simulink model "Test2_2"  (R2021a)
(part 3 of 3)

  Line 71 : spsDistributedParametersLineLib/Distributed Parameters Line  Phases=3  Length=0.16999  Frequency=50  Resistance=[0.646656091154803 0.0486237908083191 0.0486712220507153;0.0486237908083191 0.646561225344642 0.0486237934466192;0.0486712220507153 0.0486237934466192 0.646656091154803]  Inductance=[0.00282448912315926 0.00133270803418135 0.00132951476746136;0.00133270803418135 0.00282479813276775 0.00133799988507366;0.00132951476746136 0.00133799988507366 0.00282448912315926]  Capacitance=[7.89543174552926e-09 -1.85986777702161e-09 -1.7901190036642e-09;-1.85986777702161e-09 7.82540023894543e-09 -1.8957321828871e-09;-1.7901190036642e-09 -1.8957321828871e-09 7.91264394645417e-09]  x1=[130.230707636067 9966.01246212464 9965.41426921905;314.159265358979 314.159265358979 314.159265358979;1.01292996287477 -0.183692598773052 -1.7546536630313]  x2=[130.231666358781 9965.86534817877 9965.2673720638;314.159265358979 314.159265358979 314.159265358979;1.01293460745813 -0.183698024049707 -1.75465903275388]  x3=[0.11680712246644 24.2072409105011 24.4001350687789;314.159265358979 314.159265358979 314.159265358979;0.99559201404185 -0.16833311922206 -1.73942871924422]  x4=[0.110940912518223 26.5128987572226 26.7063295888185;314.159265358979 314.159265358979 314.159265358979;1.03092689690365 -0.197915914084497 -1.76876362475642]  x5=8.14502446416769e-07  V1=ones(3,3)  V2=ones(3,3)  I1=ones(3,3)  I2=ones(3,3)  nHarmo=1  Measurements=None  Decoupling=off  VsMag0=0  VrMag0=0  VsAngle0=0  VrAngle0=0  IsMag0=0  IrMag0=0  IsAngle0=0  IrAngle0=0
      settings: SourceProductBaseCode=PS
  Line 72 : spsDistributedParametersLineLib/Distributed Parameters Line  Phases=3  Length=0.27999  Frequency=50  Resistance=[0.646656091154803 0.0486237908083191 0.0486712220507153;0.0486237908083191 0.646561225344642 0.0486237934466192;0.0486712220507153 0.0486237934466192 0.646656091154803]  Inductance=[0.00282448912315926 0.00133270803418135 0.00132951476746136;0.00133270803418135 0.00282479813276775 0.00133799988507366;0.00132951476746136 0.00133799988507366 0.00282448912315926]  Capacitance=[7.89543174552926e-09 -1.85986777702161e-09 -1.7901190036642e-09;-1.85986777702161e-09 7.82540023894543e-09 -1.8957321828871e-09;-1.7901190036642e-09 -1.8957321828871e-09 7.91264394645417e-09]  x1=[130.081348911455 9976.99844767141 9976.35824041174;314.159265358979 314.159265358979 314.159265358979;1.01268721771526 -0.183283432469296 -1.75424455593335]  x2=[130.230707636067 9966.01246212464 9965.41426921905;314.159265358979 314.159265358979 314.159265358979;1.01276438146455 -0.183824142328408 -1.75478533180681]  x3=[0.351945699224796 33.0670710232444 32.8199427170776;314.159265358979 314.159265358979 314.159265358979;0.207747752541117 2.58745975030086 1.0223784525399]  x4=[0.254167918835229 82.4346919282585 82.619054469803;314.159265358979 314.159265358979 314.159265358979;2.64798945434631 -0.329445271930397 -1.89678242777258]  x5=1.341564444804e-06  V1=ones(3,3)  V2=ones(3,3)  I1=ones(3,3)  I2=ones(3,3)  nHarmo=1  Measurements=None  Decoupling=off  VsMag0=0  VrMag0=0  VsAngle0=0  VrAngle0=0  IsMag0=0  IrMag0=0  IsAngle0=0  IrAngle0=0
      settings: SourceProductBaseCode=PS
  Line 73 : spsDistributedParametersLineLib/Distributed Parameters Line  Phases=3  Length=0.01  Frequency=50  Resistance=[0.646656091154803 0.0486237908083191 0.0486712220507153;0.0486237908083191 0.646561225344642 0.0486237934466192;0.0486712220507153 0.0486237934466192 0.646656091154803]  Inductance=[0.00282448912315926 0.00133270803418135 0.00132951476746136;0.00133270803418135 0.00282479813276775 0.00133799988507366;0.00132951476746136 0.00133799988507366 0.00282448912315926]  Capacitance=[7.89543174552926e-09 -1.85986777702161e-09 -1.7901190036642e-09;-1.85986777702161e-09 7.82540023894543e-09 -1.8957321828871e-09;-1.7901190036642e-09 -1.8957321828871e-09 7.91264394645417e-09]  x1=[130.076014067588 9977.39085152671 9976.74914367271;314.159265358979 314.159265358979 314.159265358979;1.01309087195348 -0.182941272422882 -1.75390208607958]  x2=[130.081348911455 9976.9984476714 9976.35824041174;314.159265358979 314.159265358979 314.159265358979;1.0130936297602 -0.182960564791928 -1.75392138090882]  x3=[0.351978223037803 33.0705703263258 32.8233930888697;314.159265358979 314.159265358979 314.159265358979;0.208150829615969 2.58773785503595 1.02265661264299]  x4=[0.254237413967942 82.4786371856206 82.663380177016;314.159265358979 314.159265358979 314.159265358979;2.64887893860995 -0.328802030937441 -1.89613838575731]  x5=4.79147271261115e-08  V1=ones(3,3)  V2=ones(3,3)  I1=ones(3,3)  I2=ones(3,3)  nHarmo=1  Measurements=None  Decoupling=off  VsMag0=0  VrMag0=0  VsAngle0=0  VrAngle0=0  IsMag0=0  IrMag0=0  IsAngle0=0  IrAngle0=0
      settings: SourceProductBaseCode=PS
  Line 74 : spsDistributedParametersLineLib/Distributed Parameters Line  Phases=3  Length=0.04  Frequency=50  Resistance=[0.646656091154803 0.0486237908083191 0.0486712220507153;0.0486237908083191 0.646561225344642 0.0486237934466192;0.0486712220507153 0.0486237934466192 0.646656091154803]  Inductance=[0.00282448912315926 0.00133270803418135 0.00132951476746136;0.00133270803418135 0.00282479813276775 0.00133799988507366;0.00132951476746136 0.00133799988507366 0.00282448912315926]  Capacitance=[7.89543174552926e-09 -1.85986777702161e-09 -1.7901190036642e-09;-1.85986777702161e-09 7.82540023894543e-09 -1.8957321828871e-09;-1.7901190036642e-09 -1.8957321828871e-09 7.91264394645417e-09]  x1=[130.054674407228 9978.96048980824 9978.31277955769;314.159265358979 314.159265358979 314.159265358979;1.01303468087487 -0.182899991815375 -1.75386082971175]  x2=[130.076014067588 9977.39085152672 9976.74914367271;314.159265358979 314.159265358979 314.159265358979;1.01304571338706 -0.182977147937979 -1.75393799574563]  x3=[0.351967320325577 33.0666328859275 32.8194352751504;314.159265358979 314.159265358979 314.159265358979;0.208050372349346 2.58764038125158 1.02255895809718]  x4=[0.254236673448409 82.4773408673841 82.6620672276254;314.159265358979 314.159265358979 314.159265358979;2.6488539053286 -0.328827139194275 -1.89616350237567]  x5=1.91658908504446e-07  V1=ones(3,3)  V2=ones(3,3)  I1=ones(3,3)  I2=ones(3,3)  nHarmo=1  Measurements=None  Decoupling=off  VsMag0=0  VrMag0=0  VsAngle0=0  VrAngle0=0  IsMag0=0  IrMag0=0  IsAngle0=0  IrAngle0=0
      settings: SourceProductBaseCode=PS
  Line 75 : spsDistributedParametersLineLib/Distributed Parameters Line  Phases=3  Length=0.23  Frequency=50  Resistance=[0.646656091154803 0.0486237908083191 0.0486712220507153;0.0486237908083191 0.646561225344642 0.0486237934466192;0.0486712220507153 0.0486237934466192 0.646656091154803]  Inductance=[0.00282448912315926 0.00133270803418135 0.00132951476746136;0.00133270803418135 0.00282479813276775 0.00133799988507366;0.00132951476746136 0.00133799988507366 0.00282448912315926]  Capacitance=[7.89543174552926e-09 -1.85986777702161e-09 -1.7901190036642e-09;-1.85986777702161e-09 7.82540023894543e-09 -1.8957321828871e-09;-1.7901190036642e-09 -1.8957321828871e-09 7.91264394645417e-09]  x1=[132.412260404274 9804.45058362649 9804.44542068226;314.159265358979 314.159265358979 314.159265358979;1.01400079471883 -0.191512094576426 -1.76247536456498]  x2=[132.463644567909 9800.85070742944 9800.85908991131;314.159265358979 314.159265358979 314.159265358979;1.01403095544799 -0.191682957837417 -1.76264642626444]  x3=[0.201444563725322 5.91804966428605 5.9047215966924;314.159265358979 314.159265358979 314.159265358979;0.461275939437241 0.877082063076161 -0.728437900325085]  x4=[0.121619568555495 47.317972952253 47.5167935580992;314.159265358979 314.159265358979 314.159265358979;2.06777818856542 -0.301596093803467 -1.86970736913679]  x5=1.10203872390056e-06  V1=ones(3,3)  V2=ones(3,3)  I1=ones(3,3)  I2=ones(3,3)  nHarmo=1  Measurements=None  Decoupling=off  VsMag0=0  VrMag0=0  VsAngle0=0  VrAngle0=0  IsMag0=0  IrMag0=0  IsAngle0=0  IrAngle0=0
      settings: SourceProductBaseCode=PS
  Line 76 : spsDistributedParametersLineLib/Distributed Parameters Line  Phases=3  Length=1.62  Frequency=50  Resistance=[0.80718830189013 0.0486237908083191 0.0486712220507153;0.0486237908083191 0.807093436079969 0.0486237934466192;0.0486712220507153 0.0486237934466192 0.80718830189013]  Inductance=[0.00279786707424938 0.00133270803418135 0.00132951476746136;0.00133270803418135 0.00279817608385787 0.00133799988507366;0.00132951476746136 0.00133799988507366 0.00279786707424938]  Capacitance=[7.73340098830622e-09 -1.79942827973291e-09 -1.73218055098733e-09;-1.79942827973291e-09 7.66505189233746e-09 -1.83375898618858e-09;-1.73218055098733e-09 -1.83375898618858e-09 7.749673531177e-09]  x1=[55.945966993339 9804.5358454258 9804.6105183802;314.159265358979 314.159265358979 314.159265358979;1.07738009221999 -0.197446923817235 -1.76837194176404]  x2=[55.9463733224315 9804.53267731463 9804.60740490844;314.159265358979 314.159265358979 314.159265358979;1.07738098322596 -0.197450312552494 -1.76837534864892]  x3=[0.048782988865129 24.8163020226173 25.0053176417309;314.159265358979 314.159265358979 314.159265358979;1.07397701542993 -0.199145104328598 -1.77007334483569]  x4=[0.0486344229699074 24.8439993842728 25.0330218787076;314.159265358979 314.159265358979 314.159265358979;1.07836957224309 -0.197652494246344 -1.76857592031423]  x5=7.70442045759223e-06  V1=ones(3,3)  V2=ones(3,3)  I1=ones(3,3)  I2=ones(3,3)  nHarmo=1  Measurements=None  Decoupling=off  VsMag0=0  VrMag0=0  VsAngle0=0  VrAngle0=0  IsMag0=0  IrMag0=0  IsAngle0=0  IrAngle0=0
      settings: SourceProductBaseCode=PS
  Line 77 : spsDistributedParametersLineLib/Distributed Parameters Line  Phases=3  Length=0.54002  Frequency=50  Resistance=[0.646656091154803 0.0486237908083191 0.0486712220507153;0.0486237908083191 0.646561225344642 0.0486237934466192;0.0486712220507153 0.0486237934466192 0.646656091154803]  Inductance=[0.00282448912315926 0.00133270803418135 0.00132951476746136;0.00133270803418135 0.00282479813276775 0.00133799988507366;0.00132951476746136 0.00133799988507366 0.00282448912315926]  Capacitance=[7.89543174552926e-09 -1.85986777702161e-09 -1.7901190036642e-09;-1.85986777702161e-09 7.82540023894543e-09 -1.8957321828871e-09;-1.7901190036642e-09 -1.8957321828871e-09 7.91264394645417e-09]  x1=[132.291266816328 9812.89477090012 9812.85777166442;314.159265358979 314.159265358979 314.159265358979;1.01346404772917 -0.191480026465655 -1.76244316834521]  x2=[132.412260404274 9804.45058362648 9804.44542068226;314.159265358979 314.159265358979 314.159265358979;1.01353412609343 -0.191882832149439 -1.76284645505391]  x3=[0.201567889892652 5.87666255876112 5.86393316817952;314.159265358979 314.159265358979 314.159265358979;0.458951197067185 0.872065549478006 -0.733742805316799]  x4=[0.121849735716523 47.3209732619761 47.5197600194276;314.159265358979 314.159265358979 314.159265358979;2.06926877558048 -0.300800439731374 -1.86890738882715]  x5=2.58749109426427e-06  V1=ones(3,3)  V2=ones(3,3)  I1=ones(3,3)  I2=ones(3,3)  nHarmo=1  Measurements=None  Decoupling=off  VsMag0=0  VrMag0=0  VsAngle0=0  VrAngle0=0  IsMag0=0  IrMag0=0  IsAngle0=0  IrAngle0=0
      settings: SourceProductBaseCode=PS
  Line 78 : spsDistributedParametersLineLib/Distributed Parameters Line  Phases=3  Length=0.13998  Frequency=50  Resistance=[0.646656091154803 0.0486237908083191 0.0486712220507153;0.0486237908083191 0.646561225344642 0.0486237934466192;0.0486712220507153 0.0486237934466192 0.646656091154803]  Inductance=[0.00282448912315926 0.00133270803418135 0.00132951476746136;0.00133270803418135 0.00282479813276775 0.00133799988507366;0.00132951476746136 0.00133799988507366 0.00282448912315926]  Capacitance=[7.89543174552926e-09 -1.85986777702161e-09 -1.7901190036642e-09;-1.85986777702161e-09 7.82540023894543e-09 -1.8957321828871e-09;-1.7901190036642e-09 -1.8957321828871e-09 7.91264394645417e-09]  x1=[132.291266816328 9812.89477090012 9812.85777166442;314.159265358979 314.159265358979 314.159265358979;1.01406622215955 -0.191001638430341 -1.76196432491836]  x2=[132.292845424718 9812.66004338261 9812.62343176244;314.159265358979 314.159265358979 314.159265358979;1.01407237967124 -0.191008438249104 -1.76197103940269]  x3=[0.12096739474067 22.8643419842892 23.0551762295825;314.159265358979 314.159265358979 314.159265358979;0.978461634859785 -0.153044666068339 -1.7243421085877]  x4=[0.110511651176818 27.1030634556416 27.2952571420408;314.159265358979 314.159265358979 314.159265358979;1.05282682069514 -0.223180765740182 -1.79390083466488]  x5=6.70710350311308e-07  V1=ones(3,3)  V2=ones(3,3)  I1=ones(3,3)  I2=ones(3,3)  nHarmo=1  Measurements=None  Decoupling=off  VsMag0=0  VrMag0=0  VsAngle0=0  VrAngle0=0  IsMag0=0  IrMag0=0  IsAngle0=0  IrAngle0=0
      settings: SourceProductBaseCode=PS
  Line 79 : spsDistributedParametersLineLib/Distributed Parameters Line  Phases=3  Length=0.14997  Frequency=50  Resistance=[0.476003738225748 0.351747138225748 0.351747138225748;0.351747138225748 0.476003738225748 0.351747138225748;0.351747138225748 0.351747138225748 0.476003738225748]  Inductance=[0.000705954362986426 0.000459934243504405 0.000459934243504405;0.000459934243504405 0.000705954362986426 0.000459934243504405;0.000459934243504405 0.000459934243504405 0.000705954362986426]  Capacitance=[5.7561313269996e-07 -1.37543883484145e-07 -1.37543912800485e-07;-1.37543883484145e-07 5.75613027339387e-07 -1.37543875208088e-07;-1.37543912800485e-07 -1.37543875208088e-07 5.75613005057695e-07]  x1=[4.71515960684011 9813.69450340501 9814.51176058105;314.159265358979 314.159265358979 314.159265358979;1.25450518806029 -0.109813676620328 -1.68063059343959]  x2=[4.71516216671498 9813.64296638232 9814.4602192662;314.159265358979 314.159265358979 314.159265358979;1.2545039381504 -0.109814213858509 -1.68063113067772]  x3=[0.0639907956313669 525.855364885648 525.899115869334;314.159265358979 314.159265358979 314.159265358979;1.25346387218607 -0.108157208623661 -1.67897412521659]  x4=[0.0639907219423131 530.093106739202 530.137210630382;314.159265358979 314.159265358979 314.159265358979;1.25450319439072 -0.112079167068294 -1.68289608406262]  x5=3.31498451375949e-06  V1=ones(3,3)  V2=ones(3,3)  I1=ones(3,3)  I2=ones(3,3)  nHarmo=1  Measurements=None  Decoupling=off  VsMag0=0  VrMag0=0  VsAngle0=0  VrAngle0=0  IsMag0=0  IrMag0=0  IsAngle0=0  IrAngle0=0
      settings: SourceProductBaseCode=PS
  Line 8 : spsDistributedParametersLineLib/Distributed Parameters Line  Phases=3  Length=0.54002  Frequency=50  Resistance=[0.646656091154803 0.0486237908083191 0.0486712220507153;0.0486237908083191 0.646561225344642 0.0486237934466192;0.0486712220507153 0.0486237934466192 0.646656091154803]  Inductance=[0.00282448912315926 0.00133270803418135 0.00132951476746136;0.00133270803418135 0.00282479813276775 0.00133799988507366;0.00132951476746136 0.00133799988507366 0.00282448912315926]  Capacitance=[7.89543174552926e-09 -1.85986777702161e-09 -1.7901190036642e-09;-1.85986777702161e-09 7.82540023894543e-09 -1.8957321828871e-09;-1.7901190036642e-09 -1.8957321828871e-09 7.91264394645417e-09]  x1=[131.737607363178 9850.69941802642 9850.17864308144;314.159265358979 314.159265358979 314.159265358979;1.06906824241826 2.25892076126052 -2.45322280325767]  x2=[131.749735782929 9848.86865393328 9848.36073374528;314.159265358979 314.159265358979 314.159265358979;1.06911835002861 2.25882438625055 -2.45331782899078]  x3=[0.126165540353935 20.1433647221107 20.3624969468267;314.159265358979 314.159265358979 314.159265358979;1.00194096644596 2.30506910238496 -2.40791035448599]  x4=[0.104769515257823 29.9954148200453 30.1573900029457;314.159265358979 314.159265358979 314.159265358979;1.14909044449937 2.22731573734265 -2.48443339458061]  x5=2.58749109426427e-06  V1=ones(3,3)  V2=ones(3,3)  I1=ones(3,3)  I2=ones(3,3)  nHarmo=1  Measurements=None  Decoupling=off  VsMag0=0  VrMag0=0  VsAngle0=0  VrAngle0=0  IsMag0=0  IrMag0=0  IsAngle0=0  IrAngle0=0
      settings: SourceProductBaseCode=PS
  Line 80 : spsDistributedParametersLineLib/Distributed Parameters Line  Phases=3  Length=0.50001  Frequency=50  Resistance=[0.646656091154803 0.0486237908083191 0.0486712220507153;0.0486237908083191 0.646561225344642 0.0486237934466192;0.0486712220507153 0.0486237934466192 0.646656091154803]  Inductance=[0.00282448912315926 0.00133270803418135 0.00132951476746136;0.00133270803418135 0.00282479813276775 0.00133799988507366;0.00132951476746136 0.00133799988507366 0.00282448912315926]  Capacitance=[7.89543174552926e-09 -1.85986777702161e-09 -1.7901190036642e-09;-1.85986777702161e-09 7.82540023894543e-09 -1.8957321828871e-09;-1.7901190036642e-09 -1.8957321828871e-09 7.91264394645417e-09]  x1=[132.173511194652 9821.5491506484 9821.48128373896;314.159265358979 314.159265358979 314.159265358979;1.0134375447102 -0.191035064587028 -1.76199801385489]  x2=[132.291266816328 9812.89477090012 9812.85777166442;314.159265358979 314.159265358979 314.159265358979;1.01352427420392 -0.191432180487021 -1.76239527682059]  x3=[0.208251616174679 6.04681336924297 5.95781439739661;314.159265358979 314.159265358979 314.159265358979;0.454006047704687 1.25385757439675 -0.347831363027163]  x4=[0.123233192274608 49.5472322137343 49.745025795091;314.159265358979 314.159265358979 314.159265358979;2.12459359899353 -0.312913395507311 -1.88108383764282]  x5=2.3957842710327e-06  V1=ones(3,3)  V2=ones(3,3)  I1=ones(3,3)  I2=ones(3,3)  nHarmo=1  Measurements=None  Decoupling=off  VsMag0=0  VrMag0=0  VsAngle0=0  VrAngle0=0  IsMag0=0  IrMag0=0  IsAngle0=0  IrAngle0=0
      settings: SourceProductBaseCode=PS
  Line 81 : spsDistributedParametersLineLib/Distributed Parameters Line  Phases=3  Length=0.17  Frequency=50  Resistance=[0.646656091154803 0.0486237908083191 0.0486712220507153;0.0486237908083191 0.646561225344642 0.0486237934466192;0.0486712220507153 0.0486237934466192 0.646656091154803]  Inductance=[0.00282448912315926 0.00133270803418135 0.00132951476746136;0.00133270803418135 0.00282479813276775 0.00133799988507366;0.00132951476746136 0.00133799988507366 0.00282448912315926]  Capacitance=[7.89543174552926e-09 -1.85986777702161e-09 -1.7901190036642e-09;-1.85986777702161e-09 7.82540023894543e-09 -1.8957321828871e-09;-1.7901190036642e-09 -1.8957321828871e-09 7.91264394645417e-09]  x1=[132.173511194652 9821.5491506484 9821.48128373896;314.159265358979 314.159265358979 314.159265358979;1.01393430399369 -0.190640421962455 -1.76160299555848]  x2=[132.174611034258 9821.39203565152 9821.32452928868;314.159265358979 314.159265358979 314.159265358979;1.01393658179971 -0.190641437142496 -1.76160396248969]  x3=[0.117821532066125 23.996687820586 24.1879409451263;314.159265358979 314.159265358979 314.159265358979;0.990089624694144 -0.161975456637961 -1.73317290655121]  x4=[0.113355728035019 26.0018361630863 26.1938777560759;314.159265358979 314.159265358979 314.159265358979;1.03845993908498 -0.217290771556384 -1.78805201032636]  x5=8.14550361143895e-07  V1=ones(3,3)  V2=ones(3,3)  I1=ones(3,3)  I2=ones(3,3)  nHarmo=1  Measurements=None  Decoupling=off  VsMag0=0  VrMag0=0  VsAngle0=0  VrAngle0=0  IsMag0=0  IrMag0=0  IsAngle0=0  IrAngle0=0
      settings: SourceProductBaseCode=PS
  Line 82 : spsDistributedParametersLineLib/Distributed Parameters Line  Phases=3  Length=0.27998  Frequency=50  Resistance=[0.646656091154803 0.0486237908083191 0.0486712220507153;0.0486237908083191 0.646561225344642 0.0486237934466192;0.0486712220507153 0.0486237934466192 0.646656091154803]  Inductance=[0.00282448912315926 0.00133270803418135 0.00132951476746136;0.00133270803418135 0.00282479813276775 0.00133799988507366;0.00132951476746136 0.00133799988507366 0.00282448912315926]  Capacitance=[7.89543174552926e-09 -1.85986777702161e-09 -1.7901190036642e-09;-1.85986777702161e-09 7.82540023894543e-09 -1.8957321828871e-09;-1.7901190036642e-09 -1.8957321828871e-09 7.91264394645417e-09]  x1=[132.105723330459 9826.65273155558 9826.56698331564;314.159265358979 314.159265358979 314.159265358979;1.01371649706855 -0.190547975485568 -1.76151066831513]  x2=[132.173511194652 9821.5491506484 9821.48128373896;314.159265358979 314.159265358979 314.159265358979;1.01376875268919 -0.190771941600801 -1.76173464039421]  x3=[0.211636496235117 6.68880111407065 6.57085313286914;314.159265358979 314.159265358979 314.159265358979;0.448331216526076 1.41419172603944 -0.182002646191028]  x4=[0.124839280490729 50.6584149883052 50.8552864090743;314.159265358979 314.159265358979 314.159265358979;2.15192808628306 -0.323173368600227 -1.89135406139734]  x5=1.34151653007687e-06  V1=ones(3,3)  V2=ones(3,3)  I1=ones(3,3)  I2=ones(3,3)  nHarmo=1  Measurements=None  Decoupling=off  VsMag0=0  VrMag0=0  VsAngle0=0  VrAngle0=0  IsMag0=0  IrMag0=0  IsAngle0=0  IrAngle0=0
      settings: SourceProductBaseCode=PS
  Line 83 : spsDistributedParametersLineLib/Distributed Parameters Line  Phases=3  Length=0.03  Frequency=50  Resistance=[0.476003738225748 0.351747138225748 0.351747138225748;0.351747138225748 0.476003738225748 0.351747138225748;0.351747138225748 0.351747138225748 0.476003738225748]  Inductance=[0.000705954362986426 0.000459934243504405 0.000459934243504405;0.000459934243504405 0.000705954362986426 0.000459934243504405;0.000459934243504405 0.000459934243504405 0.000705954362986426]  Capacitance=[5.7561313269996e-07 -1.37543883484145e-07 -1.37543912800485e-07;-1.37543883484145e-07 5.75613027339387e-07 -1.37543875208088e-07;-1.37543912800485e-07 -1.37543875208088e-07 5.75613005057695e-07]  x1=[5.70282059813818 9777.61614892348 9777.73874302418;314.159265358979 314.159265358979 314.159265358979;1.28263867287871 2.17477579081481 -2.53751546513187]  x2=[5.70282402151544 9777.6163039351 9777.73889895204;314.159265358979 314.159265358979 314.159265358979;1.28263665860042 2.17477576530025 -2.53751549074301]  x3=[0.0774700274359414 526.350277214598 526.356899317948;314.159265358979 314.159265358979 314.159265358979;1.27855129628944 2.17458627167104 -2.53770554021627]  x4=[0.0775438111432303 526.350340456895 526.35683612321;314.159265358979 314.159265358979 314.159265358979;1.28651189534568 2.17484043953016 -2.53745026053335]  x5=6.63129528657629e-07  V1=ones(3,3)  V2=ones(3,3)  I1=ones(3,3)  I2=ones(3,3)  nHarmo=1  Measurements=None  Decoupling=off  VsMag0=0  VrMag0=0  VsAngle0=0  VrAngle0=0  IsMag0=0  IrMag0=0  IsAngle0=0  IrAngle0=0
      settings: SourceProductBaseCode=PS
  Line 84 : spsDistributedParametersLineLib/Distributed Parameters Line  Phases=3  Length=0.02  Frequency=50  Resistance=[0.646656091154803 0.0486237908083191 0.0486712220507153;0.0486237908083191 0.646561225344642 0.0486237934466192;0.0486712220507153 0.0486237934466192 0.646656091154803]  Inductance=[0.00282448912315926 0.00133270803418135 0.00132951476746136;0.00133270803418135 0.00282479813276775 0.00133799988507366;0.00132951476746136 0.00133799988507366 0.00282448912315926]  Capacitance=[7.89543174552926e-09 -1.85986777702161e-09 -1.7901190036642e-09;-1.85986777702161e-09 7.82540023894543e-09 -1.8957321828871e-09;-1.7901190036642e-09 -1.8957321828871e-09 7.91264394645417e-09]  x1=[132.789126266165 9781.02683598408 9780.42031592206;314.159265358979 314.159265358979 314.159265358979;1.0694910373007 2.25677854886239 -2.45535788755353]  x2=[132.789137662631 9781.02358008288 9780.417064447;314.159265358979 314.159265358979 314.159265358979;1.06949120331148 2.25677843562566 -2.45535799936825]  x3=[0.116761225704046 24.6778683791443 24.8674778921864;314.159265358979 314.159265358979 314.159265358979;1.06907973129993 2.25980703976288 -2.45234982662511]  x4=[0.115440893096846 25.1044925257125 25.2941175783022;314.159265358979 314.159265358979 314.159265358979;1.06987693711702 2.25377769785739 -2.45833905984952]  x5=9.5829454252223e-08  V1=ones(3,3)  V2=ones(3,3)  I1=ones(3,3)  I2=ones(3,3)  nHarmo=1  Measurements=None  Decoupling=off  VsMag0=0  VrMag0=0  VsAngle0=0  VrAngle0=0  IsMag0=0  IrMag0=0  IsAngle0=0  IrAngle0=0
      settings: SourceProductBaseCode=PS
  Line 85 : spsDistributedParametersLineLib/Distributed Parameters Line  Phases=3  Length=0.5  Frequency=50  Resistance=[0.646656091154803 0.0486237908083191 0.0486712220507153;0.0486237908083191 0.646561225344642 0.0486237934466192;0.0486712220507153 0.0486237934466192 0.646656091154803]  Inductance=[0.00282448912315926 0.00133270803418135 0.00132951476746136;0.00133270803418135 0.00282479813276775 0.00133799988507366;0.00132951476746136 0.00133799988507366 0.00282448912315926]  Capacitance=[7.89543174552926e-09 -1.85986777702161e-09 -1.7901190036642e-09;-1.85986777702161e-09 7.82540023894543e-09 -1.8957321828871e-09;-1.7901190036642e-09 -1.8957321828871e-09 7.91264394645417e-09]  x1=[132.772277667242 9782.18789453562 9781.57741920365;314.159265358979 314.159265358979 314.159265358979;1.06865004930001 2.25627362822203 -2.45586345652191]  x2=[132.789126266165 9781.02683598408 9780.42031592206;314.159265358979 314.159265358979 314.159265358979;1.06876850023796 2.25620454062084 -2.45593244221029]  x3=[0.138932344380155 21.3879588893918 21.5760908704784;314.159265358979 314.159265358979 314.159265358979;0.997328465291815 2.27881622397395 -2.43417244694111]  x4=[0.0940686620565523 28.3796934758062 28.569767773675;314.159265358979 314.159265358979 314.159265358979;1.17330576576078 2.23870042108029 -2.47282996263106]  x5=2.39573635630557e-06  V1=ones(3,3)  V2=ones(3,3)  I1=ones(3,3)  I2=ones(3,3)  nHarmo=1  Measurements=None  Decoupling=off  VsMag0=0  VrMag0=0  VsAngle0=0  VrAngle0=0  IsMag0=0  IrMag0=0  IsAngle0=0  IrAngle0=0
      settings: SourceProductBaseCode=PS
  Line 86 : spsDistributedParametersLineLib/Distributed Parameters Line  Phases=3  Length=0.23  Frequency=50  Resistance=[0.646656091154803 0.0486237908083191 0.0486712220507153;0.0486237908083191 0.646561225344642 0.0486237934466192;0.0486712220507153 0.0486237934466192 0.646656091154803]  Inductance=[0.00282448912315926 0.00133270803418135 0.00132951476746136;0.00133270803418135 0.00282479813276775 0.00133799988507366;0.00132951476746136 0.00133799988507366 0.00282448912315926]  Capacitance=[7.89543174552926e-09 -1.85986777702161e-09 -1.7901190036642e-09;-1.85986777702161e-09 7.82540023894543e-09 -1.8957321828871e-09;-1.7901190036642e-09 -1.8957321828871e-09 7.91264394645417e-09]  x1=[132.763119314431 9783.00719565047 9782.39424411809;314.159265358979 314.159265358979 314.159265358979;1.06899046178697 2.25663045801336 -2.4555064707107]  x2=[132.772277667242 9782.18789453562 9781.57741920365;314.159265358979 314.159265358979 314.159265358979;1.06905647639781 2.2565965078579 -2.45554026952749]  x3=[0.143597106193202 20.0832952923519 20.2705925459986;314.159265358979 314.159265358979 314.159265358979;0.98901855645717 2.32630530774299 -2.38715277073359]  x4=[0.0897348029105246 29.7768464771282 29.9663998686376;314.159265358979 314.159265358979 314.159265358979;1.19681358000998 2.20939971113767 -2.50198336508607]  x5=1.10203872390056e-06  V1=ones(3,3)  V2=ones(3,3)  I1=ones(3,3)  I2=ones(3,3)  nHarmo=1  Measurements=None  Decoupling=off  VsMag0=0  VrMag0=0  VsAngle0=0  VrAngle0=0  IsMag0=0  IrMag0=0  IsAngle0=0  IrAngle0=0
      settings: SourceProductBaseCode=PS
  Line 87 : spsDistributedParametersLineLib/Distributed Parameters Line  Phases=3  Length=1.62  Frequency=50  Resistance=[0.80718830189013 0.0486237908083191 0.0486712220507153;0.0486237908083191 0.807093436079969 0.0486237934466192;0.0486712220507153 0.0486237934466192 0.80718830189013]  Inductance=[0.00279786707424938 0.00133270803418135 0.00132951476746136;0.00133270803418135 0.00279817608385787 0.00133799988507366;0.00132951476746136 0.00133799988507366 0.00279786707424938]  Capacitance=[7.73340098830622e-09 -1.79942827973291e-09 -1.73218055098733e-09;-1.79942827973291e-09 7.66505189233746e-09 -1.83375898618858e-09;-1.73218055098733e-09 -1.83375898618858e-09 7.749673531177e-09]  x1=[56.3393685664166 9783.09162793975 9782.56182202606;314.159265358979 314.159265358979 314.159265358979;1.02643034834768 2.25931904448646 -2.45285760389577]  x2=[56.3398015731102 9783.08191094594 9782.55218276093;314.159265358979 314.159265358979 314.159265358979;1.02643301251892 2.25931608136779 -2.45286058287975]  x3=[0.0491576657452382 24.7596318145718 24.9466956947032;314.159265358979 314.159265358979 314.159265358979;1.02319452565439 2.25781599346474 -2.45436505584523]  x4=[0.0489447535654206 24.7920310467614 24.9790941839298;314.159265358979 314.159265358979 314.159265358979;1.02725646422453 2.25891888154773 -2.45325499695565]  x5=7.70442045759223e-06  V1=ones(3,3)  V2=ones(3,3)  I1=ones(3,3)  I2=ones(3,3)  nHarmo=1  Measurements=None  Decoupling=off  VsMag0=0  VrMag0=0  VsAngle0=0  VrAngle0=0  IsMag0=0  IrMag0=0  IsAngle0=0  IrAngle0=0
      settings: SourceProductBaseCode=PS
  Line 88 : spsDistributedParametersLineLib/Distributed Parameters Line  Phases=3  Length=0.54002  Frequency=50  Resistance=[0.646656091154803 0.0486237908083191 0.0486712220507153;0.0486237908083191 0.646561225344642 0.0486237934466192;0.0486712220507153 0.0486237934466192 0.646656091154803]  Inductance=[0.00282448912315926 0.00133270803418135 0.00132951476746136;0.00133270803418135 0.00282479813276775 0.00133799988507366;0.00132951476746136 0.00133799988507366 0.00282448912315926]  Capacitance=[7.89543174552926e-09 -1.85986777702161e-09 -1.7901190036642e-09;-1.85986777702161e-09 7.82540023894543e-09 -1.8957321828871e-09;-1.7901190036642e-09 -1.8957321828871e-09 7.91264394645417e-09]  x1=[132.741273272324 9784.92376829306 9784.30496184118;314.159265358979 314.159265358979 314.159265358979;1.06836945341264 2.25634143966523 -2.45579618398973]  x2=[132.763119314431 9783.00719565047 9782.39424411809;314.159265358979 314.159265358979 314.159265358979;1.06852379316157 2.25625972044035 -2.45587756119963]  x3=[0.143641248405531 20.0607836635622 20.248008773117;314.159265358979 314.159265358979 314.159265358979;0.98583218030511 2.32343330437969 -2.39002868167626]  x4=[0.0897014943316794 29.7831134823281 29.9725499420936;314.159265358979 314.159265358979 314.159265358979;1.19991552005365 2.21056085927069 -2.50081763905518]  x5=2.58749109426427e-06  V1=ones(3,3)  V2=ones(3,3)  I1=ones(3,3)  I2=ones(3,3)  nHarmo=1  Measurements=None  Decoupling=off  VsMag0=0  VrMag0=0  VsAngle0=0  VrAngle0=0  IsMag0=0  IrMag0=0  IsAngle0=0  IrAngle0=0
      settings: SourceProductBaseCode=PS
  Line 89 : spsDistributedParametersLineLib/Distributed Parameters Line  Phases=3  Length=0.13998  Frequency=50  Resistance=[0.646656091154803 0.0486237908083191 0.0486712220507153;0.0486237908083191 0.646561225344642 0.0486237934466192;0.0486712220507153 0.0486237934466192 0.646656091154803]  Inductance=[0.00282448912315926 0.00133270803418135 0.00132951476746136;0.00133270803418135 0.00282479813276775 0.00133799988507366;0.00132951476746136 0.00133799988507366 0.00282448912315926]  Capacitance=[7.89543174552926e-09 -1.85986777702161e-09 -1.7901190036642e-09;-1.85986777702161e-09 7.82540023894543e-09 -1.8957321828871e-09;-1.7901190036642e-09 -1.8957321828871e-09 7.91264394645417e-09]  x1=[132.741273272324 9784.92376829306 9784.30496184118;314.159265358979 314.159265358979 314.159265358979;1.06897162784302 2.25681982770054 -2.45531734056288]  x2=[132.742144181348 9784.70157324549 9784.08312046605;314.159265358979 314.159265358979 314.159265358979;1.06898234819054 2.25681364423754 -2.45532343075775]  x3=[0.122348512607476 22.9207989995043 23.1102774805994;314.159265358979 314.159265358979 314.159265358979;1.06151645242125 2.29351332151557 -2.41889675270657]  x4=[0.109764101877681 26.9025028907462 27.0920681426183;314.159265358979 314.159265358979 314.159265358979;1.07707009525723 2.22539834880836 -2.48654410911055]  x5=6.70710350311308e-07  V1=ones(3,3)  V2=ones(3,3)  I1=ones(3,3)  I2=ones(3,3)  nHarmo=1  Measurements=None  Decoupling=off  VsMag0=0  VrMag0=0  VsAngle0=0  VrAngle0=0  IsMag0=0  IrMag0=0  IsAngle0=0  IrAngle0=0
      settings: SourceProductBaseCode=PS
  Line 9 : spsDistributedParametersLineLib/Distributed Parameters Line  Phases=3  Length=0.13998  Frequency=50  Resistance=[0.646656091154803 0.0486237908083191 0.0486712220507153;0.0486237908083191 0.646561225344642 0.0486237934466192;0.0486712220507153 0.0486237934466192 0.646656091154803]  Inductance=[0.00282448912315926 0.00133270803418135 0.00132951476746136;0.00133270803418135 0.00282479813276775 0.00133799988507366;0.00132951476746136 0.00133799988507366 0.00282448912315926]  Capacitance=[7.89543174552926e-09 -1.85986777702161e-09 -1.7901190036642e-09;-1.85986777702161e-09 7.82540023894543e-09 -1.8957321828871e-09;-1.7901190036642e-09 -1.8957321828871e-09 7.91264394645417e-09]  x1=[131.737607363178 9850.69941802642 9850.17864308144;314.159265358979 314.159265358979 314.159265358979;1.06967041684863 2.25939914929583 -2.45274395983082]  x2=[131.738146099414 9850.54058868395 9850.0200090178;314.159265358979 314.159265358979 314.159265358979;1.06967879000639 2.25939310066086 -2.4527499382122]  x3=[0.119847205487519 23.5509521578462 23.7419853359846;314.159265358979 314.159265358979 314.159265358979;1.06772903623956 2.27977439156491 -2.43251296261474]  x4=[0.110503582508618 26.5878301855748 26.779037154267;314.159265358979 314.159265358979 314.159265358979;1.07156505501998 2.24118790525267 -2.4708439643076]  x5=6.70710350311308e-07  V1=ones(3,3)  V2=ones(3,3)  I1=ones(3,3)  I2=ones(3,3)  nHarmo=1  Measurements=None  Decoupling=off  VsMag0=0  VrMag0=0  VsAngle0=0  VrAngle0=0  IsMag0=0  IrMag0=0  IsAngle0=0  IrAngle0=0
      settings: SourceProductBaseCode=PS
  Line 90 : spsDistributedParametersLineLib/Distributed Parameters Line  Phases=3  Length=0.14997  Frequency=50  Resistance=[0.476003738225748 0.351747138225748 0.351747138225748;0.351747138225748 0.476003738225748 0.351747138225748;0.351747138225748 0.351747138225748 0.476003738225748]  Inductance=[0.000705954362986426 0.000459934243504405 0.000459934243504405;0.000459934243504405 0.000705954362986426 0.000459934243504405;0.000459934243504405 0.000459934243504405 0.000705954362986426]  Capacitance=[5.7561313269996e-07 -1.37543883484145e-07 -1.37543912800485e-07;-1.37543883484145e-07 5.75613027339387e-07 -1.37543875208088e-07;-1.37543912800485e-07 -1.37543875208088e-07 5.75613005057695e-07]  x1=[3.62838796694639 9851.63719589281 9851.85858599348;314.159265358979 314.159265358979 314.159265358979;1.30289632755562 2.17728914964739 -2.53500824297292]  x2=[3.62838993117416 9851.60136193109 9851.82275122619;314.159265358979 314.159265358979 314.159265358979;1.30289507320158 2.17728859167297 -2.53500880094729]  x3=[0.0492418432482476 528.498059284221 528.509894969357;314.159265358979 314.159265358979 314.159265358979;1.30185368891968 2.17820493731586 -2.53409245513826]  x4=[0.0492419064510967 531.532638855963 531.544542736239;314.159265358979 314.159265358979 314.159265358979;1.30289564998328 2.17575559094808 -2.53654180178885]  x5=3.31498451375949e-06  V1=ones(3,3)  V2=ones(3,3)  I1=ones(3,3)  I2=ones(3,3)  nHarmo=1  Measurements=None  Decoupling=off  VsMag0=0  VrMag0=0  VsAngle0=0  VrAngle0=0  IsMag0=0  IrMag0=0  IsAngle0=0  IrAngle0=0
      settings: SourceProductBaseCode=PS
  Line 91 : spsDistributedParametersLineLib/Distributed Parameters Line  Phases=3  Length=0.50001  Frequency=50  Resistance=[0.646656091154803 0.0486237908083191 0.0486712220507153;0.0486237908083191 0.646561225344642 0.0486237934466192;0.0486712220507153 0.0486237934466192 0.646656091154803]  Inductance=[0.00282448912315926 0.00133270803418135 0.00132951476746136;0.00133270803418135 0.00282479813276775 0.00133799988507366;0.00132951476746136 0.00133799988507366 0.00282448912315926]  Capacitance=[7.89543174552926e-09 -1.85986777702161e-09 -1.7901190036642e-09;-1.85986777702161e-09 7.82540023894543e-09 -1.8957321828871e-09;-1.7901190036642e-09 -1.8957321828871e-09 7.91264394645417e-09]  x1=[131.72436565465 9852.95782936429 9852.42444400894;314.159265358979 314.159265358979 314.159265358979;1.0690524409797 2.25907994193154 -2.45306507192224]  x2=[131.737607363178 9850.69941802642 9850.17864308144;314.159265358979 314.159265358979 314.159265358979;1.06912846889301 2.25896860723915 -2.45317491173305]  x3=[0.130839345427691 18.6625362785029 18.881067013325;314.159265358979 314.159265358979 314.159265358979;1.00188876918853 2.33388258016365 -2.37947862946837]  x4=[0.100132534653049 31.5363417717655 31.6982649736186;314.159265358979 314.159265358979 314.159265358979;1.15607831111184 2.21427597413681 -2.49743613497584]  x5=2.3957842710327e-06  V1=ones(3,3)  V2=ones(3,3)  I1=ones(3,3)  I2=ones(3,3)  nHarmo=1  Measurements=None  Decoupling=off  VsMag0=0  VrMag0=0  VsAngle0=0  VrAngle0=0  IsMag0=0  IrMag0=0  IsAngle0=0  IrAngle0=0
      settings: SourceProductBaseCode=PS
  Line 92 : spsDistributedParametersLineLib/Distributed Parameters Line  Phases=3  Length=0.17  Frequency=50  Resistance=[0.646656091154803 0.0486237908083191 0.0486712220507153;0.0486237908083191 0.646561225344642 0.0486237934466192;0.0486712220507153 0.0486237934466192 0.646656091154803]  Inductance=[0.00282448912315926 0.00133270803418135 0.00132951476746136;0.00133270803418135 0.00282479813276775 0.00133799988507366;0.00132951476746136 0.00133799988507366 0.00282448912315926]  Capacitance=[7.89543174552926e-09 -1.85986777702161e-09 -1.7901190036642e-09;-1.85986777702161e-09 7.82540023894543e-09 -1.8957321828871e-09;-1.7901190036642e-09 -1.8957321828871e-09 7.91264394645417e-09]  x1=[131.72436565465 9852.95782936429 9852.42444400894;314.159265358979 314.159265358979 314.159265358979;1.06954920026319 2.25947458455612 -2.45267005362583]  x2=[131.72470187884 9852.82734590794 9852.29405478689;314.159265358979 314.159265358979 314.159265358979;1.06955685319491 2.25946763519511 -2.4526769405039]  x3=[0.118483746040794 23.9499619906877 24.1410016374452;314.159265358979 314.159265358979 314.159265358979;1.07182009354702 2.26802289386471 -2.44417671274052]  x4=[0.111840622195946 26.1910875959685 26.382330507613;314.159265358979 314.159265358979 314.159265358979;1.06688779436018 2.25145649393546 -2.46064327253397]  x5=8.14550361143895e-07  V1=ones(3,3)  V2=ones(3,3)  I1=ones(3,3)  I2=ones(3,3)  nHarmo=1  Measurements=None  Decoupling=off  VsMag0=0  VrMag0=0  VsAngle0=0  VrAngle0=0  IsMag0=0  IrMag0=0  IsAngle0=0  IrAngle0=0
      settings: SourceProductBaseCode=PS
  Line 93 : spsDistributedParametersLineLib/Distributed Parameters Line  Phases=3  Length=0.27999  Frequency=50  Resistance=[0.646656091154803 0.0486237908083191 0.0486712220507153;0.0486237908083191 0.646561225344642 0.0486237934466192;0.0486712220507153 0.0486237934466192 0.646656091154803]  Inductance=[0.00282448912315926 0.00133270803418135 0.00132951476746136;0.00133270803418135 0.00282479813276775 0.00133799988507366;0.00132951476746136 0.00133799988507366 0.00282448912315926]  Capacitance=[7.89543174552926e-09 -1.85986777702161e-09 -1.7901190036642e-09;-1.85986777702161e-09 7.82540023894543e-09 -1.8957321828871e-09;-1.7901190036642e-09 -1.8957321828871e-09 7.91264394645417e-09]  x1=[131.716357672896 9854.43556321463 9853.89495614932;314.159265358979 314.159265358979 314.159265358979;1.06932857856634 2.25941705894742 -2.45272864192755]  x2=[131.72436565465 9852.95782936429 9852.42444400894;314.159265358979 314.159265358979 314.159265358979;1.06938363390584 2.25934305295927 -2.45280171043145]  x3=[0.134146287528651 17.5710391978824 17.7892016664237;314.159265358979 314.159265358979 314.159265358979;1.00547334515192 2.35013464511156 -2.36348460092551]  x4=[0.0968066198216025 32.6776398271596 32.83972593296;314.159265358979 314.159265358979 314.159265358979;1.15743161522017 2.21037101750281 -2.50134093851114]  x5=1.341564444804e-06  V1=ones(3,3)  V2=ones(3,3)  I1=ones(3,3)  I2=ones(3,3)  nHarmo=1  Measurements=None  Decoupling=off  VsMag0=0  VrMag0=0  VsAngle0=0  VrAngle0=0  IsMag0=0  IrMag0=0  IsAngle0=0  IrAngle0=0
      settings: SourceProductBaseCode=PS
  Line 94 : spsDistributedParametersLineLib/Distributed Parameters Line  Phases=3  Length=0.28003  Frequency=50  Resistance=[0.476003738225748 0.351747138225748 0.351747138225748;0.351747138225748 0.476003738225748 0.351747138225748;0.351747138225748 0.351747138225748 0.476003738225748]  Inductance=[0.000705954362986426 0.000459934243504405 0.000459934243504405;0.000459934243504405 0.000705954362986426 0.000459934243504405;0.000459934243504405 0.000459934243504405 0.000705954362986426]  Capacitance=[5.7561313269996e-07 -1.37543883484145e-07 -1.37543912800485e-07;-1.37543883484145e-07 5.75613027339387e-07 -1.37543875208088e-07;-1.37543912800485e-07 -1.37543875208088e-07 5.75613005057695e-07]  x1=[3.80334430622162 9843.2740131217 9843.523656068;314.159265358979 314.159265358979 314.159265358979;1.31995517931882 2.17625289329607 -2.53603870136241]  x2=[3.80337031493527 9843.28123557039 9843.53088466247;314.159265358979 314.159265358979 314.159265358979;1.31993116900823 2.17625171350132 -2.53603988179229]  x3=[0.0515020769120263 529.220891178604 529.234315488892;314.159265358979 314.159265358979 314.159265358979;1.31391436133396 2.1750399480961 -2.53725203611312]  x4=[0.0515707878976852 529.220934271935 529.234272799149;314.159265358979 314.159265358979 314.159265358979;1.324018462075 2.17629882744582 -2.53599237810464]  x5=6.18987206366653e-06  V1=ones(3,3)  V2=ones(3,3)  I1=ones(3,3)  I2=ones(3,3)  nHarmo=1  Measurements=None  Decoupling=off  VsMag0=0  VrMag0=0  VsAngle0=0  VrAngle0=0  IsMag0=0  IrMag0=0  IsAngle0=0  IrAngle0=0
      settings: SourceProductBaseCode=PS
  Line 95 : spsDistributedParametersLineLib/Distributed Parameters Line  Phases=3  Length=1.11  Frequency=50  Resistance=[0.502970710632245 0.0486237908083191 0.0486712220507153;0.0486237908083191 0.502875844822084 0.0486237934466192;0.0486712220507153 0.0486237934466192 0.502970710632245]  Inductance=[0.00286900545038753 0.00133270803418135 0.00132951476746136;0.00133270803418135 0.00286931445999602 0.00133799988507366;0.00132951476746136 0.00133799988507366 0.00286900545038753]  Capacitance=[8.11484299003193e-09 -1.94249816214699e-09 -1.86930692621136e-09;-1.94249816214699e-09 8.0425699231653e-09 -1.98049571960044e-09;-1.86930692621136e-09 -1.98049571960044e-09 8.13337738722527e-09]  x1=[235.972722765501 9823.60661442259 9823.63166873049;314.159265358979 314.159265358979 314.159265358979;0.992400204045535 -0.186638763463349 -1.75764462186215]  x2=[235.973059211092 9823.61580103942 9823.64087605943;314.159265358979 314.159265358979 314.159265358979;0.992399711834075 -0.186639641265451 -1.7576455072254]  x3=[0.206875609901839 24.9891343751895 25.1810719572439;314.159265358979 314.159265358979 314.159265358979;0.990711301617362 -0.188006796455805 -1.75901419770931]  x4=[0.206875609937 24.9891343826934 25.1810719648655;314.159265358979 314.159265358979 314.159265358979;0.992399711824948 -0.186639641265194 -1.75764550722568]  x5=5.37516004033389e-06  V1=ones(3,3)  V2=ones(3,3)  I1=ones(3,3)  I2=ones(3,3)  nHarmo=1  Measurements=None  Decoupling=off  VsMag0=0  VrMag0=0  VsAngle0=0  VrAngle0=0  IsMag0=0  IrMag0=0  IsAngle0=0  IrAngle0=0
      settings: SourceProductBaseCode=PS
  Line 96 : spsDistributedParametersLineLib/Distributed Parameters Line  Phases=3  Length=0.02  Frequency=50  Resistance=[0.646656091154803 0.0486237908083191 0.0486712220507153;0.0486237908083191 0.646561225344642 0.0486237934466192;0.0486712220507153 0.0486237934466192 0.646656091154803]  Inductance=[0.00282448912315926 0.00133270803418135 0.00132951476746136;0.00133270803418135 0.00282479813276775 0.00133799988507366;0.00132951476746136 0.00133799988507366 0.00282448912315926]  Capacitance=[7.89543174552926e-09 -1.85986777702161e-09 -1.7901190036642e-09;-1.85986777702161e-09 7.82540023894543e-09 -1.8957321828871e-09;-1.7901190036642e-09 -1.8957321828871e-09 7.91264394645417e-09]  x1=[132.238781069031 9824.24966881278 9824.42365326744;314.159265358979 314.159265358979 314.159265358979;1.01407673318113 -0.191434581799565 -1.7624130275415]  x2=[132.238913203071 9824.23295491704 9824.40694442497;314.159265358979 314.159265358979 314.159265358979;1.01407760316247 -0.191436146854563 -1.7624145850362]  x3=[0.119849524113915 23.5126032193936 23.704750034429;314.159265358979 314.159265358979 314.159265358979;0.997200693981198 -0.196369622194781 -1.76736696540049]  x4=[0.11142568066128 26.4900246158514 26.6828148190489;314.159265358979 314.159265358979 314.159265358979;1.03219840414421 -0.187078283168997 -1.75803607624414]  x5=9.5829454252223e-08  V1=ones(3,3)  V2=ones(3,3)  I1=ones(3,3)  I2=ones(3,3)  nHarmo=1  Measurements=None  Decoupling=off  VsMag0=0  VrMag0=0  VsAngle0=0  VrAngle0=0  IsMag0=0  IrMag0=0  IsAngle0=0  IrAngle0=0
      settings: SourceProductBaseCode=PS
  Line 97 : spsDistributedParametersLineLib/Distributed Parameters Line  Phases=3  Length=1.15  Frequency=50  Resistance=[0.646656091154803 0.0486237908083191 0.0486712220507153;0.0486237908083191 0.646561225344642 0.0486237934466192;0.0486712220507153 0.0486237934466192 0.646656091154803]  Inductance=[0.00282448912315926 0.00133270803418135 0.00132951476746136;0.00133270803418135 0.00282479813276775 0.00133799988507366;0.00132951476746136 0.00133799988507366 0.00282448912315926]  Capacitance=[7.89543174552926e-09 -1.85986777702161e-09 -1.7901190036642e-09;-1.85986777702161e-09 7.82540023894543e-09 -1.8957321828871e-09;-1.7901190036642e-09 -1.8957321828871e-09 7.91264394645417e-09]  x1=[132.238781069031 9824.24966881277 9824.42365326744;314.159265358979 314.159265358979 314.159265358979;1.01237576051259 -0.192785892868221 -1.76376562496261]  x2=[132.249103184869 9822.80452364585 9822.98060352948;314.159265358979 314.159265358979 314.159265358979;1.0124193439274 -0.192846062930569 -1.76382526131069]  x3=[0.119954314263027 23.2582073273627 23.4496015134105;314.159265358979 314.159265358979 314.159265358979;0.983726702076203 -0.172481104376235 -1.74367143064433]  x4=[0.111263697286357 26.685453073985 26.8778727073974;314.159265358979 314.159265358979 314.159265358979;1.041509442515 -0.211826369759663 -1.78264163825617]  x5=5.51019361950282e-06  V1=ones(3,3)  V2=ones(3,3)  I1=ones(3,3)  I2=ones(3,3)  nHarmo=1  Measurements=None  Decoupling=off  VsMag0=0  VrMag0=0  VsAngle0=0  VrAngle0=0  IsMag0=0  IrMag0=0  IsAngle0=0  IrAngle0=0
      settings: SourceProductBaseCode=PS
  Line 98 : spsDistributedParametersLineLib/Distributed Parameters Line  Phases=3  Length=0.18999  Frequency=50  Resistance=[0.646656091154803 0.0486237908083191 0.0486712220507153;0.0486237908083191 0.646561225344642 0.0486237934466192;0.0486712220507153 0.0486237934466192 0.646656091154803]  Inductance=[0.00282448912315926 0.00133270803418135 0.00132951476746136;0.00133270803418135 0.00282479813276775 0.00133799988507366;0.00132951476746136 0.00133799988507366 0.00282448912315926]  Capacitance=[7.89543174552926e-09 -1.85986777702161e-09 -1.7901190036642e-09;-1.85986777702161e-09 7.82540023894543e-09 -1.8957321828871e-09;-1.7901190036642e-09 -1.8957321828871e-09 7.91264394645417e-09]  x1=[132.249103184869 9822.80452364585 9822.98060352948;314.159265358979 314.159265358979 314.159265358979;1.01386443310574 -0.191698034488958 -1.7626761400273]  x2=[132.249598083623 9822.72722935742 9822.90338710963;314.159265358979 314.159265358979 314.159265358979;1.01386736446996 -0.19170203426094 -1.76268010762714]  x3=[0.117171906433535 24.4042106065448 24.5964138696598;314.159265358979 314.159265358979 314.159265358979;1.00651389056184 -0.187029071322245 -1.75805143318559]  x4=[0.114073339542497 25.5812193822577 25.7737439431915;314.159265358979 314.159265358979 314.159265358979;1.02112773040748 -0.19637807063123 -1.76731570630407]  x5=9.10331900668992e-07  V1=ones(3,3)  V2=ones(3,3)  I1=ones(3,3)  I2=ones(3,3)  nHarmo=1  Measurements=None  Decoupling=off  VsMag0=0  VrMag0=0  VsAngle0=0  VrAngle0=0  IsMag0=0  IrMag0=0  IsAngle0=0  IrAngle0=0
      settings: SourceProductBaseCode=PS
  Line 99 : spsDistributedParametersLineLib/Distributed Parameters Line  Phases=3  Length=0.34002  Frequency=50  Resistance=[0.646656091154803 0.0486237908083191 0.0486712220507153;0.0486237908083191 0.646561225344642 0.0486237934466192;0.0486712220507153 0.0486237934466192 0.646656091154803]  Inductance=[0.00282448912315926 0.00133270803418135 0.00132951476746136;0.00133270803418135 0.00282479813276775 0.00133799988507366;0.00132951476746136 0.00133799988507366 0.00282448912315926]  Capacitance=[7.89543174552926e-09 -1.85986777702161e-09 -1.7901190036642e-09;-1.85986777702161e-09 7.82540023894543e-09 -1.8957321828871e-09;-1.7901190036642e-09 -1.8957321828871e-09 7.91264394645417e-09]  x1=[132.249103184869 9822.80452364585 9822.98060352948;314.159265358979 314.159265358979 314.159265358979;1.01363859511507 -0.191877447939958 -1.7628557242672]  x2=[132.251183868736 9822.51156326851 9822.6881155278;314.159265358979 314.159265358979 314.159265358979;1.01364651316723 -0.191887563396408 -1.76286573506996]  x3=[0.118435175027337 23.8634990245014 24.0554005303904;314.159265358979 314.159265358979 314.159265358979;0.993577001546536 -0.175414285646175 -1.74654720079815]  x4=[0.112836028738313 26.1186268387006 26.3112601488089;314.159265358979 314.159265358979 314.159265358979;1.03417938239328 -0.207317823663926 -1.7781650691274]  x5=1.62919655174204e-06  V1=ones(3,3)  V2=ones(3,3)  I1=ones(3,3)  I2=ones(3,3)  nHarmo=1  Measurements=None  Decoupling=off  VsMag0=0  VrMag0=0  VsAngle0=0  VrAngle0=0  IsMag0=0  IrMag0=0  IsAngle0=0  IrAngle0=0
      settings: SourceProductBaseCode=PS
  Line im1 : spsDistributedParametersLineLib/Distributed Parameters Line  Phases=3  Length=1e-10  Frequency=50  Resistance=[0.646656091154803 0.0486237908083191 0.0486712220507153;0.0486237908083191 0.646561225344642 0.0486237934466192;0.0486712220507153 0.0486237934466192 0.646656091154803]  Inductance=[0.00282448912315926 0.00133270803418135 0.00132951476746136;0.00133270803418135 0.00282479813276775 0.00133799988507366;0.00132951476746136 0.00133799988507366 0.00282448912315926]  Capacitance=[7.89543174552926e-09 -1.85986777702161e-09 -1.7901190036642e-09;-1.85986777702161e-09 7.82540023894543e-09 -1.8957321828871e-09;-1.7901190036642e-09 -1.8957321828871e-09 7.91264394645417e-09]  x1=[131.708950173583 9855.73083509479 9855.1889775783;314.159265358979 314.159265358979 314.159265358979;1.06977044630333 2.25982353745412 -2.45232222251488]  x2=[131.708950173592 9855.73083509355 9855.18897757707;314.159265358979 314.159265358979 314.159265358979;1.06977044630333 2.25982353745404 -2.45232222251496]  x3=[0.143498641314375 6.5800375689919 6.8561671898256;314.159265358979 314.159265358979 314.159265358979;0.590898553232277 2.61598483652511 -2.1261574755364]  x4=[0.110351014969903 44.0433903706656 44.0797608432614;314.159265358979 314.159265358979 314.159265358979;1.50155951426119 2.20772162154927 -2.50181020878131]  x5=4.79147271261115e-16  V1=ones(3,3)  V2=ones(3,3)  I1=ones(3,3)  I2=ones(3,3)  nHarmo=1  Measurements=None  Decoupling=off  VsMag0=0  VrMag0=0  VsAngle0=0  VrAngle0=0  IsMag0=0  IrMag0=0  IsAngle0=0  IrAngle0=0
      settings: SourceProductBaseCode=PS
  Line im2 : spsDistributedParametersLineLib/Distributed Parameters Line  Phases=3  Length=1e-10  Frequency=50  Resistance=[0.646656091154803 0.0486237908083191 0.0486712220507153;0.0486237908083191 0.646561225344642 0.0486237934466192;0.0486712220507153 0.0486237934466192 0.646656091154803]  Inductance=[0.00282448912315926 0.00133270803418135 0.00132951476746136;0.00133270803418135 0.00282479813276775 0.00133799988507366;0.00132951476746136 0.00133799988507366 0.00282448912315926]  Capacitance=[7.89543174552926e-09 -1.85986777702161e-09 -1.7901190036642e-09;-1.85986777702161e-09 7.82540023894543e-09 -1.8957321828871e-09;-1.7901190036642e-09 -1.8957321828871e-09 7.91264394645417e-09]  x1=[132.622916358163 9790.14137890445 9790.19164885648;314.159265358979 314.159265358979 314.159265358979;1.01445602169012 -0.191941288685564 -1.76290542388567]  x2=[132.622916358188 9790.14137890304 9790.19164885507;314.159265358979 314.159265358979 314.159265358979;1.01445602169019 -0.191941288685634 -1.76290542388574]  x3=[0.240524169719142 6.37116443174942 6.49375905471762;314.159265358979 314.159265358979 314.159265358979;0.605727683617002 0.543183009398457 -1.03708372797203]  x4=[0.0989328394354935 45.2981759867367 45.5581804038003;314.159265358979 314.159265358979 314.159265358979;2.20711218805767 -0.286618270512059 -1.85732950037919]  x5=4.79147271261115e-16  V1=ones(3,3)  V2=ones(3,3)  I1=ones(3,3)  I2=ones(3,3)  nHarmo=1  Measurements=None  Decoupling=off  VsMag0=0  VrMag0=0  VsAngle0=0  VrAngle0=0  IsMag0=0  IrMag0=0  IsAngle0=0  IrAngle0=0
      settings: SourceProductBaseCode=PS
  Line im3 : spsDistributedParametersLineLib/Distributed Parameters Line  Phases=3  Length=1e-10  Frequency=50  Resistance=[0.646656091154803 0.0486237908083191 0.0486712220507153;0.0486237908083191 0.646561225344642 0.0486237934466192;0.0486712220507153 0.0486237934466192 0.646656091154803]  Inductance=[0.00282448912315926 0.00133270803418135 0.00132951476746136;0.00133270803418135 0.00282479813276775 0.00133799988507366;0.00132951476746136 0.00133799988507366 0.00282448912315926]  Capacitance=[7.89543174552926e-09 -1.85986777702161e-09 -1.7901190036642e-09;-1.85986777702161e-09 7.82540023894543e-09 -1.8957321828871e-09;-1.7901190036642e-09 -1.8957321828871e-09 7.91264394645417e-09]  x1=[131.273424847562 9891.53592488655 9891.23316090909;314.159265358979 314.159265358979 314.159265358979;1.013597336061 -0.187226632991791 -1.75818947616188]  x2=[131.273424847613 9891.535924883 9891.23316090554;314.159265358979 314.159265358979 314.159265358979;1.01359733606107 -0.187226632991971 -1.75818947616207]  x3=[0.343332874946799 27.9763304368335 28.0391728357135;314.159265358979 314.159265358979 314.159265358979;0.283747211489709 2.57210773422898 1.01721591298762]  x4=[0.238926437550154 76.9899079743265 77.5492590280155;314.159265358979 314.159265358979 314.159265358979;2.76760427386886 -0.323129976971323 -1.88820368513762]  x5=4.79147271261115e-16  V1=ones(3,3)  V2=ones(3,3)  I1=ones(3,3)  I2=ones(3,3)  nHarmo=1  Measurements=None  Decoupling=off  VsMag0=0  VrMag0=0  VsAngle0=0  VrAngle0=0  IsMag0=0  IrMag0=0  IsAngle0=0  IrAngle0=0
      settings: SourceProductBaseCode=PS
  Line im4 : spsDistributedParametersLineLib/Distributed Parameters Line  Phases=3  Length=1e-10  Frequency=50  Resistance=[0.646656091154803 0.0486237908083191 0.0486712220507153;0.0486237908083191 0.646561225344642 0.0486237934466192;0.0486712220507153 0.0486237934466192 0.646656091154803]  Inductance=[0.00282448912315926 0.00133270803418135 0.00132951476746136;0.00133270803418135 0.00282479813276775 0.00133799988507366;0.00132951476746136 0.00133799988507366 0.00282448912315926]  Capacitance=[7.89543174552926e-09 -1.85986777702161e-09 -1.7901190036642e-09;-1.85986777702161e-09 7.82540023894543e-09 -1.8957321828871e-09;-1.7901190036642e-09 -1.8957321828871e-09 7.91264394645417e-09]  x1=[131.76794541411 9846.3421209356 9845.85604977773;314.159265358979 314.159265358979 314.159265358979;1.06998386125906 2.25932506623598 -2.45281441092072]  x2=[131.767945414107 9846.34212093538 9845.8560497775;314.159265358979 314.159265358979 314.159265358979;1.06998386125905 2.25932506623597 -2.45281441092073]  x3=[0.103093360045065 21.7448492541278 21.7862720247723;314.159265358979 314.159265358979 314.159265358979;1.18555098212564 2.27474130672236 -2.43107861529803]  x4=[0.125808568635058 28.358915016935 28.7005214977102;314.159265358979 314.159265358979 314.159265358979;0.937551292302253 2.24733469802291 -2.46885613928613]  x5=4.79147271261115e-16  V1=ones(3,3)  V2=ones(3,3)  I1=ones(3,3)  I2=ones(3,3)  nHarmo=1  Measurements=None  Decoupling=off  VsMag0=0  VrMag0=0  VsAngle0=0  VrAngle0=0  IsMag0=0  IrMag0=0  IsAngle0=0  IrAngle0=0
      settings: SourceProductBaseCode=PS
  Line im5 : spsDistributedParametersLineLib/Distributed Parameters Line  Phases=3  Length=1e-10  Frequency=50  Resistance=[0.646656091154803 0.0486237908083191 0.0486712220507153;0.0486237908083191 0.646561225344642 0.0486237934466192;0.0486712220507153 0.0486237934466192 0.646656091154803]  Inductance=[0.00282448912315926 0.00133270803418135 0.00132951476746136;0.00133270803418135 0.00282479813276775 0.00133799988507366;0.00132951476746136 0.00133799988507366 0.00282448912315926]  Capacitance=[7.89543174552926e-09 -1.85986777702161e-09 -1.7901190036642e-09;-1.85986777702161e-09 7.82540023894543e-09 -1.8957321828871e-09;-1.7901190036642e-09 -1.8957321828871e-09 7.91264394645417e-09]  x1=[132.221106036175 9826.55451502137 9826.72616066862;314.159265358979 314.159265358979 314.159265358979;1.01401770872178 -0.191263467890853 -1.76224280579293]  x2=[132.22110603618 9826.55451502118 9826.72616066843;314.159265358979 314.159265358979 314.159265358979;1.01401770872179 -0.19126346789087 -1.76224280579294]  x3=[0.134814616689869 21.6822100466278 21.9604801307745;314.159265358979 314.159265358979 314.159265358979;0.786204522589779 -0.196912011104217 -1.77235416441796]  x4=[0.103719574094615 28.3208476713449 28.4279999769936;314.159265358979 314.159265358979 314.159265358979;1.31662137547723 -0.187100273956115 -1.75491409859185]  x5=4.79147271261115e-16  V1=ones(3,3)  V2=ones(3,3)  I1=ones(3,3)  I2=ones(3,3)  nHarmo=1  Measurements=None  Decoupling=off  VsMag0=0  VrMag0=0  VsAngle0=0  VrAngle0=0  IsMag0=0  IrMag0=0  IsAngle0=0  IrAngle0=0
      settings: SourceProductBaseCode=PS
  Line im6 : spsDistributedParametersLineLib/Distributed Parameters Line  Phases=3  Length=1e-10  Frequency=50  Resistance=[0.646656091154803 0.0486237908083191 0.0486712220507153;0.0486237908083191 0.646561225344642 0.0486237934466192;0.0486712220507153 0.0486237934466192 0.646656091154803]  Inductance=[0.00282448912315926 0.00133270803418135 0.00132951476746136;0.00133270803418135 0.00282479813276775 0.00133799988507366;0.00132951476746136 0.00133799988507366 0.00282448912315926]  Capacitance=[7.89543174552926e-09 -1.85986777702161e-09 -1.7901190036642e-09;-1.85986777702161e-09 7.82540023894543e-09 -1.8957321828871e-09;-1.7901190036642e-09 -1.8957321828871e-09 7.91264394645417e-09]  x1=[132.797050043831 9780.50733909159 9779.90266205088;314.159265358979 314.159265358979 314.159265358979;1.06957608595771 2.25677082298583 -2.45536555737826]  x2=[132.797050043835 9780.50733909135 9779.90266205066;314.159265358979 314.159265358979 314.159265358979;1.06957608595761 2.25677082298582 -2.45536555737827]  x3=[0.0918184834977501 21.3279782123213 21.8233144050181;314.159265358979 314.159265358979 314.159265358979;0.183390836726424 2.28266246459491 -2.43321613970917]  x4=[0.171025324919407 28.4567288220818 28.3370160306132;314.159265358979 314.159265358979 314.159265358979;1.41061839604629 2.23753021389099 -2.47228436428179]  x5=4.79147271261115e-16  V1=ones(3,3)  V2=ones(3,3)  I1=ones(3,3)  I2=ones(3,3)  nHarmo=1  Measurements=None  Decoupling=off  VsMag0=0  VrMag0=0  VsAngle0=0  VrAngle0=0  IsMag0=0  IrMag0=0  IsAngle0=0  IrAngle0=0
      settings: SourceProductBaseCode=PS
  Line im7 : spsDistributedParametersLineLib/Distributed Parameters Line  Phases=3  Length=1e-10  Frequency=50  Resistance=[0.646656091154803 0.0486237908083191 0.0486712220507153;0.0486237908083191 0.646561225344642 0.0486237934466192;0.0486712220507153 0.0486237934466192 0.646656091154803]  Inductance=[0.00282448912315926 0.00133270803418135 0.00132951476746136;0.00133270803418135 0.00282479813276775 0.00133799988507366;0.00132951476746136 0.00133799988507366 0.00282448912315926]  Capacitance=[7.89543174552926e-09 -1.85986777702161e-09 -1.7901190036642e-09;-1.85986777702161e-09 7.82540023894543e-09 -1.8957321828871e-09;-1.7901190036642e-09 -1.8957321828871e-09 7.91264394645417e-09]  x1=[133.212956294535 9754.96187830601 9755.18157544808;314.159265358979 314.159265358979 314.159265358979;1.01359625483318 -0.193939154062245 -1.76491083253962]  x2=[133.212956294541 9754.96187830579 9755.18157544786;314.159265358979 314.159265358979 314.159265358979;1.01359625483312 -0.193939154062266 -1.76491083253964]  x3=[0.113063497123118 20.8795448131938 21.0643966237916;314.159265358979 314.159265358979 314.159265358979;0.526451647459102 -0.203597681701978 -1.7768060781852]  x4=[0.148500615207856 28.7455064661882 28.9621674387104;314.159265358979 314.159265358979 314.159265358979;1.33740765956018 -0.187037420023698 -1.75607754653064]  x5=4.79147271261115e-16  V1=ones(3,3)  V2=ones(3,3)  I1=ones(3,3)  I2=ones(3,3)  nHarmo=1  Measurements=None  Decoupling=off  VsMag0=0  VrMag0=0  VsAngle0=0  VrAngle0=0  IsMag0=0  IrMag0=0  IsAngle0=0  IrAngle0=0
      settings: SourceProductBaseCode=PS
  Load 1 : spsThreePhaseSeriesRLCLoadLib/Three-Phase Series RLC Load  LConnTagsString=A|B|C  Configuration=Delta  NominalVoltage=11000  Vabc=[1e3 1e3 1e3]  Vabcp=[1e3 1e3 1e3]  NominalFrequency=50  UnbalancedPower=off  ActivePower=16134.902  InductivePower=2342.4939  CapacitivePower=0  Pabc=[10e3 9e3 11e3]  QLabc=[100 90 110]  QCabc=[100 90 110]  Pabcp=[10e3 9e3 11e3]  QLabcp=[100 90 110]  QCabcp=[100 90 110]  Measurements=None  LoadType=constant Z
  Load 10 : spsThreePhaseSeriesRLCLoadLib/Three-Phase Series RLC Load  LConnTagsString=A|B|C  Configuration=Delta  NominalVoltage=11000  Vabc=[1e3 1e3 1e3]  Vabcp=[1e3 1e3 1e3]  NominalFrequency=50  UnbalancedPower=off  ActivePower=16490.5134  InductivePower=6006.2436  CapacitivePower=0  Pabc=[10e3 9e3 11e3]  QLabc=[100 90 110]  QCabc=[100 90 110]  Pabcp=[10e3 9e3 11e3]  QLabcp=[100 90 110]  QCabcp=[100 90 110]  Measurements=None  LoadType=constant Z
  Load 11 : spsThreePhaseSeriesRLCLoadLib/Three-Phase Series RLC Load  LConnTagsString=A|B|C  Configuration=Delta  NominalVoltage=11000  Vabc=[1e3 1e3 1e3]  Vabcp=[1e3 1e3 1e3]  NominalFrequency=50  UnbalancedPower=off  ActivePower=19509.119  InductivePower=10068.5153  CapacitivePower=0  Pabc=[10e3 9e3 11e3]  QLabc=[100 90 110]  QCabc=[100 90 110]  Pabcp=[10e3 9e3 11e3]  QLabcp=[100 90 110]  QCabcp=[100 90 110]  Measurements=None  LoadType=constant Z
  Load 12 : spsThreePhaseSeriesRLCLoadLib/Three-Phase Series RLC Load  LConnTagsString=A|B|C  Configuration=Delta  NominalVoltage=11000  Vabc=[1e3 1e3 1e3]  Vabcp=[1e3 1e3 1e3]  NominalFrequency=50  UnbalancedPower=off  ActivePower=15240.2095  InductivePower=3674.4442  CapacitivePower=0  Pabc=[10e3 9e3 11e3]  QLabc=[100 90 110]  QCabc=[100 90 110]  Pabcp=[10e3 9e3 11e3]  QLabcp=[100 90 110]  QCabcp=[100 90 110]  Measurements=None  LoadType=constant Z
  Load 13 : spsThreePhaseSeriesRLCLoadLib/Three-Phase Series RLC Load  LConnTagsString=A|B|C  Configuration=Delta  NominalVoltage=11000  Vabc=[1e3 1e3 1e3]  Vabcp=[1e3 1e3 1e3]  NominalFrequency=50  UnbalancedPower=off  ActivePower=9826.6108  InductivePower=6086.05  CapacitivePower=0  Pabc=[10e3 9e3 11e3]  QLabc=[100 90 110]  QCabc=[100 90 110]  Pabcp=[10e3 9e3 11e3]  QLabcp=[100 90 110]  QCabcp=[100 90 110]  Measurements=None  LoadType=constant Z
  Load 14 : spsThreePhaseSeriesRLCLoadLib/Three-Phase Series RLC Load  LConnTagsString=A|B|C  Configuration=Delta  NominalVoltage=11000  Vabc=[1e3 1e3 1e3]  Vabcp=[1e3 1e3 1e3]  NominalFrequency=50  UnbalancedPower=off  ActivePower=31652.2573  InductivePower=18541.4825  CapacitivePower=0  Pabc=[10e3 9e3 11e3]  QLabc=[100 90 110]  QCabc=[100 90 110]  Pabcp=[10e3 9e3 11e3]  QLabcp=[100 90 110]  QCabcp=[100 90 110]  Measurements=None  LoadType=constant Z
  Load 15 : spsThreePhaseSeriesRLCLoadLib/Three-Phase Series RLC Load  LConnTagsString=A|B|C  Configuration=Delta  NominalVoltage=11000  Vabc=[1e3 1e3 1e3]  Vabcp=[1e3 1e3 1e3]  NominalFrequency=50  UnbalancedPower=off  ActivePower=19304.8677  InductivePower=7769.668  CapacitivePower=0  Pabc=[10e3 9e3 11e3]  QLabc=[100 90 110]  QCabc=[100 90 110]  Pabcp=[10e3 9e3 11e3]  QLabcp=[100 90 110]  QCabcp=[100 90 110]  Measurements=None  LoadType=constant Z
  Load 16 : spsThreePhaseSeriesRLCLoadLib/Three-Phase Series RLC Load  LConnTagsString=A|B|C  Configuration=Delta  NominalVoltage=11000  Vabc=[1e3 1e3 1e3]  Vabcp=[1e3 1e3 1e3]  NominalFrequency=50  UnbalancedPower=off  ActivePower=10170.1146  InductivePower=2910.348  CapacitivePower=0  Pabc=[10e3 9e3 11e3]  QLabc=[100 90 110]  QCabc=[100 90 110]  Pabcp=[10e3 9e3 11e3]  QLabcp=[100 90 110]  QCabcp=[100 90 110]  Measurements=None  LoadType=constant Z
  Load 17 : spsThreePhaseSeriesRLCLoadLib/Three-Phase Series RLC Load  LConnTagsString=A|B|C  Configuration=Delta  NominalVoltage=11000  Vabc=[1e3 1e3 1e3]  Vabcp=[1e3 1e3 1e3]  NominalFrequency=50  UnbalancedPower=off  ActivePower=22371.4494  InductivePower=4030.5791  CapacitivePower=0  Pabc=[10e3 9e3 11e3]  QLabc=[100 90 110]  QCabc=[100 90 110]  Pabcp=[10e3 9e3 11e3]  QLabcp=[100 90 110]  QCabcp=[100 90 110]  Measurements=None  LoadType=constant Z
  Load 18 : spsThreePhaseSeriesRLCLoadLib/Three-Phase Series RLC Load  LConnTagsString=A|B|C  Configuration=Delta  NominalVoltage=11000  Vabc=[1e3 1e3 1e3]  Vabcp=[1e3 1e3 1e3]  NominalFrequency=50  UnbalancedPower=off  ActivePower=26072.4046  InductivePower=13374.6223  CapacitivePower=0  Pabc=[10e3 9e3 11e3]  QLabc=[100 90 110]  QCabc=[100 90 110]  Pabcp=[10e3 9e3 11e3]  QLabcp=[100 90 110]  QCabcp=[100 90 110]  Measurements=None  LoadType=constant Z
  Load 19 : spsThreePhaseSeriesRLCLoadLib/Three-Phase Series RLC Load  LConnTagsString=A|B|C  Configuration=Delta  NominalVoltage=11000  Vabc=[1e3 1e3 1e3]  Vabcp=[1e3 1e3 1e3]  NominalFrequency=50  UnbalancedPower=off  ActivePower=278.3696  InductivePower=116.943  CapacitivePower=0  Pabc=[10e3 9e3 11e3]  QLabc=[100 90 110]  QCabc=[100 90 110]  Pabcp=[10e3 9e3 11e3]  QLabcp=[100 90 110]  QCabcp=[100 90 110]  Measurements=None  LoadType=constant Z
  Load 2 : spsThreePhaseSeriesRLCLoadLib/Three-Phase Series RLC Load  LConnTagsString=A|B|C  Configuration=Delta  NominalVoltage=11000  Vabc=[1e3 1e3 1e3]  Vabcp=[1e3 1e3 1e3]  NominalFrequency=50  UnbalancedPower=off  ActivePower=22553.8925  InductivePower=6121.1401  CapacitivePower=0  Pabc=[10e3 9e3 11e3]  QLabc=[100 90 110]  QCabc=[100 90 110]  Pabcp=[10e3 9e3 11e3]  QLabcp=[100 90 110]  QCabcp=[100 90 110]  Measurements=None  LoadType=constant Z
  Load 20 : spsThreePhaseSeriesRLCLoadLib/Three-Phase Series RLC Load  LConnTagsString=A|B|C  Configuration=Delta  NominalVoltage=11000  Vabc=[1e3 1e3 1e3]  Vabcp=[1e3 1e3 1e3]  NominalFrequency=50  UnbalancedPower=off  ActivePower=7131.277  InductivePower=2444.3212  CapacitivePower=0  Pabc=[10e3 9e3 11e3]  QLabc=[100 90 110]  QCabc=[100 90 110]  Pabcp=[10e3 9e3 11e3]  QLabcp=[100 90 110]  QCabcp=[100 90 110]  Measurements=None  LoadType=constant Z
  Load 21 : spsThreePhaseSeriesRLCLoadLib/Three-Phase Series RLC Load  LConnTagsString=A|B|C  Configuration=Delta  NominalVoltage=11000  Vabc=[1e3 1e3 1e3]  Vabcp=[1e3 1e3 1e3]  NominalFrequency=50  UnbalancedPower=off  ActivePower=31251.0059  InductivePower=21470.572  CapacitivePower=0  Pabc=[10e3 9e3 11e3]  QLabc=[100 90 110]  QCabc=[100 90 110]  Pabcp=[10e3 9e3 11e3]  QLabcp=[100 90 110]  QCabcp=[100 90 110]  Measurements=None  LoadType=constant Z
  Load 22 : spsThreePhaseSeriesRLCLoadLib/Three-Phase Series RLC Load  LConnTagsString=A|B|C  Configuration=Delta  NominalVoltage=11000  Vabc=[1e3 1e3 1e3]  Vabcp=[1e3 1e3 1e3]  NominalFrequency=50  UnbalancedPower=off  ActivePower=4956.2749  InductivePower=1340.446  CapacitivePower=0  Pabc=[10e3 9e3 11e3]  QLabc=[100 90 110]  QCabc=[100 90 110]  Pabcp=[10e3 9e3 11e3]  QLabcp=[100 90 110]  QCabcp=[100 90 110]  Measurements=None  LoadType=constant Z
  Load 23 : spsThreePhaseSeriesRLCLoadLib/Three-Phase Series RLC Load  LConnTagsString=A|B|C  Configuration=Delta  NominalVoltage=11000  Vabc=[1e3 1e3 1e3]  Vabcp=[1e3 1e3 1e3]  NominalFrequency=50  UnbalancedPower=off  ActivePower=10840.1938  InductivePower=4171.3099  CapacitivePower=0  Pabc=[10e3 9e3 11e3]  QLabc=[100 90 110]  QCabc=[100 90 110]  Pabcp=[10e3 9e3 11e3]  QLabcp=[100 90 110]  QCabcp=[100 90 110]  Measurements=None  LoadType=constant Z
  Load 24 : spsThreePhaseSeriesRLCLoadLib/Three-Phase Series RLC Load  LConnTagsString=A|B|C  Configuration=Delta  NominalVoltage=11000  Vabc=[1e3 1e3 1e3]  Vabcp=[1e3 1e3 1e3]  NominalFrequency=50  UnbalancedPower=off  ActivePower=20656.1408  InductivePower=5546.4647  CapacitivePower=0  Pabc=[10e3 9e3 11e3]  QLabc=[100 90 110]  QCabc=[100 90 110]  Pabcp=[10e3 9e3 11e3]  QLabcp=[100 90 110]  QCabcp=[100 90 110]  Measurements=None  LoadType=constant Z
  Load 25 : spsThreePhaseSeriesRLCLoadLib/Three-Phase Series RLC Load  LConnTagsString=A|B|C  Configuration=Delta  NominalVoltage=11000  Vabc=[1e3 1e3 1e3]  Vabcp=[1e3 1e3 1e3]  NominalFrequency=50  UnbalancedPower=off  ActivePower=10751.1424  InductivePower=6306.2207  CapacitivePower=0  Pabc=[10e3 9e3 11e3]  QLabc=[100 90 110]  QCabc=[100 90 110]  Pabcp=[10e3 9e3 11e3]  QLabcp=[100 90 110]  QCabcp=[100 90 110]  Measurements=None  LoadType=constant Z
  Load 26 : spsThreePhaseSeriesRLCLoadLib/Three-Phase Series RLC Load  LConnTagsString=A|B|C  Configuration=Delta  NominalVoltage=11000  Vabc=[1e3 1e3 1e3]  Vabcp=[1e3 1e3 1e3]  NominalFrequency=50  UnbalancedPower=off  ActivePower=244.875  InductivePower=133.1434  CapacitivePower=0  Pabc=[10e3 9e3 11e3]  QLabc=[100 90 110]  QCabc=[100 90 110]  Pabcp=[10e3 9e3 11e3]  QLabcp=[100 90 110]  QCabcp=[100 90 110]  Measurements=None  LoadType=constant Z
  Load 27 : spsThreePhaseSeriesRLCLoadLib/Three-Phase Series RLC Load  LConnTagsString=A|B|C  Configuration=Delta  NominalVoltage=11000  Vabc=[1e3 1e3 1e3]  Vabcp=[1e3 1e3 1e3]  NominalFrequency=50  UnbalancedPower=off  ActivePower=19009.4557  InductivePower=8095.9702  CapacitivePower=0  Pabc=[10e3 9e3 11e3]  QLabc=[100 90 110]  QCabc=[100 90 110]  Pabcp=[10e3 9e3 11e3]  QLabcp=[100 90 110]  QCabcp=[100 90 110]  Measurements=None  LoadType=constant Z
  Load 28 : spsThreePhaseSeriesRLCLoadLib/Three-Phase Series RLC Load  LConnTagsString=A|B|C  Configuration=Delta  NominalVoltage=11000  Vabc=[1e3 1e3 1e3]  Vabcp=[1e3 1e3 1e3]  NominalFrequency=50  UnbalancedPower=off  ActivePower=4360.6047  InductivePower=3096.3359  CapacitivePower=0  Pabc=[10e3 9e3 11e3]  QLabc=[100 90 110]  QCabc=[100 90 110]  Pabcp=[10e3 9e3 11e3]  QLabcp=[100 90 110]  QCabcp=[100 90 110]  Measurements=None  LoadType=constant Z
  Load 29 : spsThreePhaseSeriesRLCLoadLib/Three-Phase Series RLC Load  LConnTagsString=A|B|C  Configuration=Delta  NominalVoltage=11000  Vabc=[1e3 1e3 1e3]  Vabcp=[1e3 1e3 1e3]  NominalFrequency=50  UnbalancedPower=off  ActivePower=25347.1187  InductivePower=4974.2554  CapacitivePower=0  Pabc=[10e3 9e3 11e3]  QLabc=[100 90 110]  QCabc=[100 90 110]  Pabcp=[10e3 9e3 11e3]  QLabcp=[100 90 110]  QCabcp=[100 90 110]  Measurements=None  LoadType=constant Z
  Load 3 : spsThreePhaseSeriesRLCLoadLib/Three-Phase Series RLC Load  LConnTagsString=A|B|C  Configuration=Delta  NominalVoltage=11000  Vabc=[1e3 1e3 1e3]  Vabcp=[1e3 1e3 1e3]  NominalFrequency=50  UnbalancedPower=off  ActivePower=31025.0528  InductivePower=4435.9334  CapacitivePower=0  Pabc=[10e3 9e3 11e3]  QLabc=[100 90 110]  QCabc=[100 90 110]  Pabcp=[10e3 9e3 11e3]  QLabcp=[100 90 110]  QCabcp=[100 90 110]  Measurements=None  LoadType=constant Z
  Load 30 : spsThreePhaseSeriesRLCLoadLib/Three-Phase Series RLC Load  LConnTagsString=A|B|C  Configuration=Delta  NominalVoltage=11000  Vabc=[1e3 1e3 1e3]  Vabcp=[1e3 1e3 1e3]  NominalFrequency=50  UnbalancedPower=off  ActivePower=4674.1639  InductivePower=1213.8354  CapacitivePower=0  Pabc=[10e3 9e3 11e3]  QLabc=[100 90 110]  QCabc=[100 90 110]  Pabcp=[10e3 9e3 11e3]  QLabcp=[100 90 110]  QCabcp=[100 90 110]  Measurements=None  LoadType=constant Z
  Load 31 : spsThreePhaseSeriesRLCLoadLib/Three-Phase Series RLC Load  LConnTagsString=A|B|C  Configuration=Delta  NominalVoltage=11000  Vabc=[1e3 1e3 1e3]  Vabcp=[1e3 1e3 1e3]  NominalFrequency=50  UnbalancedPower=off  ActivePower=7648.8189  InductivePower=2387.6308  CapacitivePower=0  Pabc=[10e3 9e3 11e3]  QLabc=[100 90 110]  QCabc=[100 90 110]  Pabcp=[10e3 9e3 11e3]  QLabcp=[100 90 110]  QCabcp=[100 90 110]  Measurements=None  LoadType=constant Z
  Load 32 : spsThreePhaseSeriesRLCLoadLib/Three-Phase Series RLC Load  LConnTagsString=A|B|C  Configuration=Delta  NominalVoltage=11000  Vabc=[1e3 1e3 1e3]  Vabcp=[1e3 1e3 1e3]  NominalFrequency=50  UnbalancedPower=off  ActivePower=20102.3771  InductivePower=8826.0815  CapacitivePower=0  Pabc=[10e3 9e3 11e3]  QLabc=[100 90 110]  QCabc=[100 90 110]  Pabcp=[10e3 9e3 11e3]  QLabcp=[100 90 110]  QCabcp=[100 90 110]  Measurements=None  LoadType=constant Z
  Load 33 : spsThreePhaseSeriesRLCLoadLib/Three-Phase Series RLC Load  LConnTagsString=A|B|C  Configuration=Delta  NominalVoltage=11000  Vabc=[1e3 1e3 1e3]  Vabcp=[1e3 1e3 1e3]  NominalFrequency=50  UnbalancedPower=off  ActivePower=8774.8348  InductivePower=3853.3526  CapacitivePower=0  Pabc=[10e3 9e3 11e3]  QLabc=[100 90 110]  QCabc=[100 90 110]  Pabcp=[10e3 9e3 11e3]  QLabcp=[100 90 110]  QCabcp=[100 90 110]  Measurements=None  LoadType=constant Z
  Load 34 : spsThreePhaseSeriesRLCLoadLib/Three-Phase Series RLC Load  LConnTagsString=A|B|C  Configuration=Delta  NominalVoltage=11000  Vabc=[1e3 1e3 1e3]  Vabcp=[1e3 1e3 1e3]  NominalFrequency=50  UnbalancedPower=off  ActivePower=249.018  InductivePower=101.5866  CapacitivePower=0  Pabc=[10e3 9e3 11e3]  QLabc=[100 90 110]  QCabc=[100 90 110]  Pabcp=[10e3 9e3 11e3]  QLabcp=[100 90 110]  QCabcp=[100 90 110]  Measurements=None  LoadType=constant Z
  Load 35 : spsThreePhaseSeriesRLCLoadLib/Three-Phase Series RLC Load  LConnTagsString=A|B|C  Configuration=Delta  NominalVoltage=11000  Vabc=[1e3 1e3 1e3]  Vabcp=[1e3 1e3 1e3]  NominalFrequency=50  UnbalancedPower=off  ActivePower=20802.1515  InductivePower=12589.8232  CapacitivePower=0  Pabc=[10e3 9e3 11e3]  QLabc=[100 90 110]  QCabc=[100 90 110]  Pabcp=[10e3 9e3 11e3]  QLabcp=[100 90 110]  QCabcp=[100 90 110]  Measurements=None  LoadType=constant Z
  Load 36 : spsThreePhaseSeriesRLCLoadLib/Three-Phase Series RLC Load  LConnTagsString=A|B|C  Configuration=Delta  NominalVoltage=11000  Vabc=[1e3 1e3 1e3]  Vabcp=[1e3 1e3 1e3]  NominalFrequency=50  UnbalancedPower=off  ActivePower=4644.8821  InductivePower=2909.8297  CapacitivePower=0  Pabc=[10e3 9e3 11e3]  QLabc=[100 90 110]  QCabc=[100 90 110]  Pabcp=[10e3 9e3 11e3]  QLabcp=[100 90 110]  QCabcp=[100 90 110]  Measurements=None  LoadType=constant Z
  Load 37 : spsThreePhaseSeriesRLCLoadLib/Three-Phase Series RLC Load  LConnTagsString=A|B|C  Configuration=Delta  NominalVoltage=11000  Vabc=[1e3 1e3 1e3]  Vabcp=[1e3 1e3 1e3]  NominalFrequency=50  UnbalancedPower=off  ActivePower=6925.4848  InductivePower=4986.3322  CapacitivePower=0  Pabc=[10e3 9e3 11e3]  QLabc=[100 90 110]  QCabc=[100 90 110]  Pabcp=[10e3 9e3 11e3]  QLabcp=[100 90 110]  QCabcp=[100 90 110]  Measurements=None  LoadType=constant Z
  Load 38 : spsThreePhaseSeriesRLCLoadLib/Three-Phase Series RLC Load  LConnTagsString=A|B|C  Configuration=Delta  NominalVoltage=11000  Vabc=[1e3 1e3 1e3]  Vabcp=[1e3 1e3 1e3]  NominalFrequency=50  UnbalancedPower=off  ActivePower=5903.135  InductivePower=3746.7294  CapacitivePower=0  Pabc=[10e3 9e3 11e3]  QLabc=[100 90 110]  QCabc=[100 90 110]  Pabcp=[10e3 9e3 11e3]  QLabcp=[100 90 110]  QCabcp=[100 90 110]  Measurements=None  LoadType=constant Z
  Load 39 : spsThreePhaseSeriesRLCLoadLib/Three-Phase Series RLC Load  LConnTagsString=A|B|C  Configuration=Delta  NominalVoltage=11000  Vabc=[1e3 1e3 1e3]  Vabcp=[1e3 1e3 1e3]  NominalFrequency=50  UnbalancedPower=off  ActivePower=9418.0557  InductivePower=5955.6281  CapacitivePower=0  Pabc=[10e3 9e3 11e3]  QLabc=[100 90 110]  QCabc=[100 90 110]  Pabcp=[10e3 9e3 11e3]  QLabcp=[100 90 110]  QCabcp=[100 90 110]  Measurements=None  LoadType=constant Z
  Load 4 : spsThreePhaseSeriesRLCLoadLib/Three-Phase Series RLC Load  LConnTagsString=A|B|C  Configuration=Delta  NominalVoltage=11000  Vabc=[1e3 1e3 1e3]  Vabcp=[1e3 1e3 1e3]  NominalFrequency=50  UnbalancedPower=off  ActivePower=29962.3434  InductivePower=7902.8743  CapacitivePower=0  Pabc=[10e3 9e3 11e3]  QLabc=[100 90 110]  QCabc=[100 90 110]  Pabcp=[10e3 9e3 11e3]  QLabcp=[100 90 110]  QCabcp=[100 90 110]  Measurements=None  LoadType=constant Z
  Load 40 : spsThreePhaseSeriesRLCLoadLib/Three-Phase Series RLC Load  LConnTagsString=A|B|C  Configuration=Delta  NominalVoltage=11000  Vabc=[1e3 1e3 1e3]  Vabcp=[1e3 1e3 1e3]  NominalFrequency=50  UnbalancedPower=off  ActivePower=4537.689  InductivePower=1671.6433  CapacitivePower=0  Pabc=[10e3 9e3 11e3]  QLabc=[100 90 110]  QCabc=[100 90 110]  Pabcp=[10e3 9e3 11e3]  QLabcp=[100 90 110]  QCabcp=[100 90 110]  Measurements=None  LoadType=constant Z
  Load 41 : spsThreePhaseSeriesRLCLoadLib/Three-Phase Series RLC Load  LConnTagsString=A|B|C  Configuration=Delta  NominalVoltage=11000  Vabc=[1e3 1e3 1e3]  Vabcp=[1e3 1e3 1e3]  NominalFrequency=50  UnbalancedPower=off  ActivePower=35020.9802  InductivePower=12301.6892  CapacitivePower=0  Pabc=[10e3 9e3 11e3]  QLabc=[100 90 110]  QCabc=[100 90 110]  Pabcp=[10e3 9e3 11e3]  QLabcp=[100 90 110]  QCabcp=[100 90 110]  Measurements=None  LoadType=constant Z
  Load 42 : spsThreePhaseSeriesRLCLoadLib/Three-Phase Series RLC Load  LConnTagsString=A|B|C  Configuration=Delta  NominalVoltage=11000  Vabc=[1e3 1e3 1e3]  Vabcp=[1e3 1e3 1e3]  NominalFrequency=50  UnbalancedPower=off  ActivePower=4911.7224  InductivePower=876.9442  CapacitivePower=0  Pabc=[10e3 9e3 11e3]  QLabc=[100 90 110]  QCabc=[100 90 110]  Pabcp=[10e3 9e3 11e3]  QLabcp=[100 90 110]  QCabcp=[100 90 110]  Measurements=None  LoadType=constant Z
  Load 43 : spsThreePhaseSeriesRLCLoadLib/Three-Phase Series RLC Load  LConnTagsString=A|B|C  Configuration=Delta  NominalVoltage=11000  Vabc=[1e3 1e3 1e3]  Vabcp=[1e3 1e3 1e3]  NominalFrequency=50  UnbalancedPower=off  ActivePower=8178.1461  InductivePower=5760.0908  CapacitivePower=0  Pabc=[10e3 9e3 11e3]  QLabc=[100 90 110]  QCabc=[100 90 110]  Pabcp=[10e3 9e3 11e3]  QLabcp=[100 90 110]  QCabcp=[100 90 110]  Measurements=None  LoadType=constant Z
  Load 44 : spsThreePhaseSeriesRLCLoadLib/Three-Phase Series RLC Load  LConnTagsString=A|B|C  Configuration=Delta  NominalVoltage=11000  Vabc=[1e3 1e3 1e3]  Vabcp=[1e3 1e3 1e3]  NominalFrequency=50  UnbalancedPower=off  ActivePower=28983.7613  InductivePower=3390.6102  CapacitivePower=0  Pabc=[10e3 9e3 11e3]  QLabc=[100 90 110]  QCabc=[100 90 110]  Pabcp=[10e3 9e3 11e3]  QLabcp=[100 90 110]  QCabcp=[100 90 110]  Measurements=None  LoadType=constant Z
  Load 45 : spsThreePhaseSeriesRLCLoadLib/Three-Phase Series RLC Load  LConnTagsString=A|B|C  Configuration=Delta  NominalVoltage=11000  Vabc=[1e3 1e3 1e3]  Vabcp=[1e3 1e3 1e3]  NominalFrequency=50  UnbalancedPower=off  ActivePower=11692.4586  InductivePower=1133.4227  CapacitivePower=0  Pabc=[10e3 9e3 11e3]  QLabc=[100 90 110]  QCabc=[100 90 110]  Pabcp=[10e3 9e3 11e3]  QLabcp=[100 90 110]  QCabcp=[100 90 110]  Measurements=None  LoadType=constant Z
  Load 46 : spsThreePhaseSeriesRLCLoadLib/Three-Phase Series RLC Load  LConnTagsString=A|B|C  Configuration=Delta  NominalVoltage=11000  Vabc=[1e3 1e3 1e3]  Vabcp=[1e3 1e3 1e3]  NominalFrequency=50  UnbalancedPower=off  ActivePower=215.6934  InductivePower=52.9262  CapacitivePower=0  Pabc=[10e3 9e3 11e3]  QLabc=[100 90 110]  QCabc=[100 90 110]  Pabcp=[10e3 9e3 11e3]  QLabcp=[100 90 110]  QCabcp=[100 90 110]  Measurements=None  LoadType=constant Z
  Load 47 : spsThreePhaseSeriesRLCLoadLib/Three-Phase Series RLC Load  LConnTagsString=A|B|C  Configuration=Delta  NominalVoltage=11000  Vabc=[1e3 1e3 1e3]  Vabcp=[1e3 1e3 1e3]  NominalFrequency=50  UnbalancedPower=off  ActivePower=18230.249  InductivePower=13465.9904  CapacitivePower=0  Pabc=[10e3 9e3 11e3]  QLabc=[100 90 110]  QCabc=[100 90 110]  Pabcp=[10e3 9e3 11e3]  QLabcp=[100 90 110]  QCabcp=[100 90 110]  Measurements=None  LoadType=constant Z
  Load 48 : spsThreePhaseSeriesRLCLoadLib/Three-Phase Series RLC Load  LConnTagsString=A|B|C  Configuration=Delta  NominalVoltage=11000  Vabc=[1e3 1e3 1e3]  Vabcp=[1e3 1e3 1e3]  NominalFrequency=50  UnbalancedPower=off  ActivePower=4366.0375  InductivePower=2795.4945  CapacitivePower=0  Pabc=[10e3 9e3 11e3]  QLabc=[100 90 110]  QCabc=[100 90 110]  Pabcp=[10e3 9e3 11e3]  QLabcp=[100 90 110]  QCabcp=[100 90 110]  Measurements=None  LoadType=constant Z
  Load 49 : spsThreePhaseSeriesRLCLoadLib/Three-Phase Series RLC Load  LConnTagsString=A|B|C  Configuration=Delta  NominalVoltage=11000  Vabc=[1e3 1e3 1e3]  Vabcp=[1e3 1e3 1e3]  NominalFrequency=50  UnbalancedPower=off  ActivePower=32216.7833  InductivePower=16649.5889  CapacitivePower=0  Pabc=[10e3 9e3 11e3]  QLabc=[100 90 110]  QCabc=[100 90 110]  Pabcp=[10e3 9e3 11e3]  QLabcp=[100 90 110]  QCabcp=[100 90 110]  Measurements=None  LoadType=constant Z
  Load 5 : spsThreePhaseSeriesRLCLoadLib/Three-Phase Series RLC Load  LConnTagsString=A|B|C  Configuration=Delta  NominalVoltage=11000  Vabc=[1e3 1e3 1e3]  Vabcp=[1e3 1e3 1e3]  NominalFrequency=50  UnbalancedPower=off  ActivePower=13704.813  InductivePower=6528.6989  CapacitivePower=0  Pabc=[10e3 9e3 11e3]  QLabc=[100 90 110]  QCabc=[100 90 110]  Pabcp=[10e3 9e3 11e3]  QLabcp=[100 90 110]  QCabcp=[100 90 110]  Measurements=None  LoadType=constant Z
  Load 50 : spsThreePhaseSeriesRLCLoadLib/Three-Phase Series RLC Load  LConnTagsString=A|B|C  Configuration=Delta  NominalVoltage=11000  Vabc=[1e3 1e3 1e3]  Vabcp=[1e3 1e3 1e3]  NominalFrequency=50  UnbalancedPower=off  ActivePower=5542.4522  InductivePower=3410.7135  CapacitivePower=0  Pabc=[10e3 9e3 11e3]  QLabc=[100 90 110]  QCabc=[100 90 110]  Pabcp=[10e3 9e3 11e3]  QLabcp=[100 90 110]  QCabcp=[100 90 110]  Measurements=None  LoadType=constant Z
  Load 51 : spsThreePhaseSeriesRLCLoadLib/Three-Phase Series RLC Load  LConnTagsString=A|B|C  Configuration=Delta  NominalVoltage=11000  Vabc=[1e3 1e3 1e3]  Vabcp=[1e3 1e3 1e3]  NominalFrequency=50  UnbalancedPower=off  ActivePower=9168.9818  InductivePower=3360.4109  CapacitivePower=0  Pabc=[10e3 9e3 11e3]  QLabc=[100 90 110]  QCabc=[100 90 110]  Pabcp=[10e3 9e3 11e3]  QLabcp=[100 90 110]  QCabcp=[100 90 110]  Measurements=None  LoadType=constant Z
  Load 52 : spsThreePhaseSeriesRLCLoadLib/Three-Phase Series RLC Load  LConnTagsString=A|B|C  Configuration=Delta  NominalVoltage=11000  Vabc=[1e3 1e3 1e3]  Vabcp=[1e3 1e3 1e3]  NominalFrequency=50  UnbalancedPower=off  ActivePower=30908.8876  InductivePower=5346.2009  CapacitivePower=0  Pabc=[10e3 9e3 11e3]  QLabc=[100 90 110]  QCabc=[100 90 110]  Pabcp=[10e3 9e3 11e3]  QLabcp=[100 90 110]  QCabcp=[100 90 110]  Measurements=None  LoadType=constant Z
  Load 53 : spsThreePhaseSeriesRLCLoadLib/Three-Phase Series RLC Load  LConnTagsString=A|B|C  Configuration=Delta  NominalVoltage=11000  Vabc=[1e3 1e3 1e3]  Vabcp=[1e3 1e3 1e3]  NominalFrequency=50  UnbalancedPower=off  ActivePower=5745.7592  InductivePower=3828.2119  CapacitivePower=0  Pabc=[10e3 9e3 11e3]  QLabc=[100 90 110]  QCabc=[100 90 110]  Pabcp=[10e3 9e3 11e3]  QLabcp=[100 90 110]  QCabcp=[100 90 110]  Measurements=None  LoadType=constant Z
  Load 54 : spsThreePhaseSeriesRLCLoadLib/Three-Phase Series RLC Load  LConnTagsString=A|B|C  Configuration=Delta  NominalVoltage=11000  Vabc=[1e3 1e3 1e3]  Vabcp=[1e3 1e3 1e3]  NominalFrequency=50  UnbalancedPower=off  ActivePower=200.7165  InductivePower=133.117  CapacitivePower=0  Pabc=[10e3 9e3 11e3]  QLabc=[100 90 110]  QCabc=[100 90 110]  Pabcp=[10e3 9e3 11e3]  QLabcp=[100 90 110]  QCabcp=[100 90 110]  Measurements=None  LoadType=constant Z
  Load 55 : spsThreePhaseSeriesRLCLoadLib/Three-Phase Series RLC Load  LConnTagsString=A|B|C  Configuration=Delta  NominalVoltage=11000  Vabc=[1e3 1e3 1e3]  Vabcp=[1e3 1e3 1e3]  NominalFrequency=50  UnbalancedPower=off  ActivePower=17407.7711  InductivePower=12566.5697  CapacitivePower=0  Pabc=[10e3 9e3 11e3]  QLabc=[100 90 110]  QCabc=[100 90 110]  Pabcp=[10e3 9e3 11e3]  QLabcp=[100 90 110]  QCabcp=[100 90 110]  Measurements=None  LoadType=constant Z
  Load 56 : spsThreePhaseSeriesRLCLoadLib/Three-Phase Series RLC Load  LConnTagsString=A|B|C  Configuration=Delta  NominalVoltage=11000  Vabc=[1e3 1e3 1e3]  Vabcp=[1e3 1e3 1e3]  NominalFrequency=50  UnbalancedPower=off  ActivePower=6906.3531  InductivePower=2528.0577  CapacitivePower=0  Pabc=[10e3 9e3 11e3]  QLabc=[100 90 110]  QCabc=[100 90 110]  Pabcp=[10e3 9e3 11e3]  QLabcp=[100 90 110]  QCabcp=[100 90 110]  Measurements=None  LoadType=constant Z
  Load 57 : spsThreePhaseSeriesRLCLoadLib/Three-Phase Series RLC Load  LConnTagsString=A|B|C  Configuration=Delta  NominalVoltage=11000  Vabc=[1e3 1e3 1e3]  Vabcp=[1e3 1e3 1e3]  NominalFrequency=50  UnbalancedPower=off  ActivePower=5944.2224  InductivePower=1977.2435  CapacitivePower=0  Pabc=[10e3 9e3 11e3]  QLabc=[100 90 110]  QCabc=[100 90 110]  Pabcp=[10e3 9e3 11e3]  QLabcp=[100 90 110]  QCabcp=[100 90 110]  Measurements=None  LoadType=constant Z
  Load 58 : spsThreePhaseSeriesRLCLoadLib/Three-Phase Series RLC Load  LConnTagsString=A|B|C  Configuration=Delta  NominalVoltage=11000  Vabc=[1e3 1e3 1e3]  Vabcp=[1e3 1e3 1e3]  NominalFrequency=50  UnbalancedPower=off  ActivePower=8725.8938  InductivePower=3535.468  CapacitivePower=0  Pabc=[10e3 9e3 11e3]  QLabc=[100 90 110]  QCabc=[100 90 110]  Pabcp=[10e3 9e3 11e3]  QLabcp=[100 90 110]  QCabcp=[100 90 110]  Measurements=None  LoadType=constant Z
  Load 59 : spsThreePhaseSeriesRLCLoadLib/Three-Phase Series RLC Load  LConnTagsString=A|B|C  Configuration=Delta  NominalVoltage=11000  Vabc=[1e3 1e3 1e3]  Vabcp=[1e3 1e3 1e3]  NominalFrequency=50  UnbalancedPower=off  ActivePower=12406.7934  InductivePower=8972.0706  CapacitivePower=0  Pabc=[10e3 9e3 11e3]  QLabc=[100 90 110]  QCabc=[100 90 110]  Pabcp=[10e3 9e3 11e3]  QLabcp=[100 90 110]  QCabcp=[100 90 110]  Measurements=None  LoadType=constant Z
  Load 6 : spsThreePhaseSeriesRLCLoadLib/Three-Phase Series RLC Load  LConnTagsString=A|B|C  Configuration=Delta  NominalVoltage=11000  Vabc=[1e3 1e3 1e3]  Vabcp=[1e3 1e3 1e3]  NominalFrequency=50  UnbalancedPower=off  ActivePower=28303.6833  InductivePower=14761.4502  CapacitivePower=0  Pabc=[10e3 9e3 11e3]  QLabc=[100 90 110]  QCabc=[100 90 110]  Pabcp=[10e3 9e3 11e3]  QLabcp=[100 90 110]  QCabcp=[100 90 110]  Measurements=None  LoadType=constant Z
  Load 60 : spsThreePhaseSeriesRLCLoadLib/Three-Phase Series RLC Load  LConnTagsString=A|B|C  Configuration=Delta  NominalVoltage=11000  Vabc=[1e3 1e3 1e3]  Vabcp=[1e3 1e3 1e3]  NominalFrequency=50  UnbalancedPower=off  ActivePower=4329.2909  InductivePower=3164.1064  CapacitivePower=0  Pabc=[10e3 9e3 11e3]  QLabc=[100 90 110]  QCabc=[100 90 110]  Pabcp=[10e3 9e3 11e3]  QLabcp=[100 90 110]  QCabcp=[100 90 110]  Measurements=None  LoadType=constant Z
  Load 7 : spsThreePhaseSeriesRLCLoadLib/Three-Phase Series RLC Load  LConnTagsString=A|B|C  Configuration=Delta  NominalVoltage=11000  Vabc=[1e3 1e3 1e3]  Vabcp=[1e3 1e3 1e3]  NominalFrequency=50  UnbalancedPower=off  ActivePower=18403.0221  InductivePower=12590.8295  CapacitivePower=0  Pabc=[10e3 9e3 11e3]  QLabc=[100 90 110]  QCabc=[100 90 110]  Pabcp=[10e3 9e3 11e3]  QLabcp=[100 90 110]  QCabcp=[100 90 110]  Measurements=None  LoadType=constant Z
  Load 8 : spsThreePhaseSeriesRLCLoadLib/Three-Phase Series RLC Load  LConnTagsString=A|B|C  Configuration=Delta  NominalVoltage=11000  Vabc=[1e3 1e3 1e3]  Vabcp=[1e3 1e3 1e3]  NominalFrequency=50  UnbalancedPower=off  ActivePower=162.2201  InductivePower=99.2001  CapacitivePower=0  Pabc=[10e3 9e3 11e3]  QLabc=[100 90 110]  QCabc=[100 90 110]  Pabcp=[10e3 9e3 11e3]  QLabcp=[100 90 110]  QCabcp=[100 90 110]  Measurements=None  LoadType=constant Z
  Load 8041 : spsThreePhaseSeriesRLCLoadLib/Three-Phase Series RLC Load  LConnTagsString=A|B|C  Configuration=Delta  NominalVoltage=11000  Vabc=[1e3 1e3 1e3]  Vabcp=[1e3 1e3 1e3]  NominalFrequency=50  UnbalancedPower=off  ActivePower=13270.2578  InductivePower=9478.9925  CapacitivePower=0  Pabc=[10e3 9e3 11e3]  QLabc=[100 90 110]  QCabc=[100 90 110]  Pabcp=[10e3 9e3 11e3]  QLabcp=[100 90 110]  QCabcp=[100 90 110]  Measurements=None  LoadType=constant Z
  Load 8173 : spsThreePhaseSeriesRLCLoadLib/Three-Phase Series RLC Load  LConnTagsString=A|B|C  Configuration=Delta  NominalVoltage=11000  Vabc=[1e3 1e3 1e3]  Vabcp=[1e3 1e3 1e3]  NominalFrequency=50  UnbalancedPower=off  ActivePower=15153.4078  InductivePower=6169.1556  CapacitivePower=0  Pabc=[10e3 9e3 11e3]  QLabc=[100 90 110]  QCabc=[100 90 110]  Pabcp=[10e3 9e3 11e3]  QLabcp=[100 90 110]  QCabcp=[100 90 110]  Measurements=None  LoadType=constant Z
  Load 8287 : spsThreePhaseSeriesRLCLoadLib/Three-Phase Series RLC Load  LConnTagsString=A|B|C  Configuration=Delta  NominalVoltage=11000  Vabc=[1e3 1e3 1e3]  Vabcp=[1e3 1e3 1e3]  NominalFrequency=50  UnbalancedPower=off  ActivePower=17355.1963  InductivePower=12915.3989  CapacitivePower=0  Pabc=[10e3 9e3 11e3]  QLabc=[100 90 110]  QCabc=[100 90 110]  Pabcp=[10e3 9e3 11e3]  QLabcp=[100 90 110]  QCabcp=[100 90 110]  Measurements=None  LoadType=constant Z
  Load 8293 : spsThreePhaseSeriesRLCLoadLib/Three-Phase Series RLC Load  LConnTagsString=A|B|C  Configuration=Delta  NominalVoltage=11000  Vabc=[1e3 1e3 1e3]  Vabcp=[1e3 1e3 1e3]  NominalFrequency=50  UnbalancedPower=off  ActivePower=6086.4676  InductivePower=4552.4157  CapacitivePower=0  Pabc=[10e3 9e3 11e3]  QLabc=[100 90 110]  QCabc=[100 90 110]  Pabcp=[10e3 9e3 11e3]  QLabcp=[100 90 110]  QCabcp=[100 90 110]  Measurements=None  LoadType=constant Z
  Load 8424 : spsThreePhaseSeriesRLCLoadLib/Three-Phase Series RLC Load  LConnTagsString=A|B|C  Configuration=Delta  NominalVoltage=11000  Vabc=[1e3 1e3 1e3]  Vabcp=[1e3 1e3 1e3]  NominalFrequency=50  UnbalancedPower=off  ActivePower=6020.7985  InductivePower=4370.761  CapacitivePower=0  Pabc=[10e3 9e3 11e3]  QLabc=[100 90 110]  QCabc=[100 90 110]  Pabcp=[10e3 9e3 11e3]  QLabcp=[100 90 110]  QCabcp=[100 90 110]  Measurements=None  LoadType=constant Z
  Load 8485 : spsThreePhaseSeriesRLCLoadLib/Three-Phase Series RLC Load  LConnTagsString=A|B|C  Configuration=Delta  NominalVoltage=11000  Vabc=[1e3 1e3 1e3]  Vabcp=[1e3 1e3 1e3]  NominalFrequency=50  UnbalancedPower=off  ActivePower=30773.7088  InductivePower=16579.4645  CapacitivePower=0  Pabc=[10e3 9e3 11e3]  QLabc=[100 90 110]  QCabc=[100 90 110]  Pabcp=[10e3 9e3 11e3]  QLabcp=[100 90 110]  QCabcp=[100 90 110]  Measurements=None  LoadType=constant Z
  Load 8551 : spsThreePhaseSeriesRLCLoadLib/Three-Phase Series RLC Load  LConnTagsString=A|B|C  Configuration=Delta  NominalVoltage=11000  Vabc=[1e3 1e3 1e3]  Vabcp=[1e3 1e3 1e3]  NominalFrequency=50  UnbalancedPower=off  ActivePower=5421.6426  InductivePower=4060.9315  CapacitivePower=0  Pabc=[10e3 9e3 11e3]  QLabc=[100 90 110]  QCabc=[100 90 110]  Pabcp=[10e3 9e3 11e3]  QLabcp=[100 90 110]  QCabcp=[100 90 110]  Measurements=None  LoadType=constant Z
  Load 8605 : spsThreePhaseSeriesRLCLoadLib/Three-Phase Series RLC Load  LConnTagsString=A|B|C  Configuration=Delta  NominalVoltage=11000  Vabc=[1e3 1e3 1e3]  Vabcp=[1e3 1e3 1e3]  NominalFrequency=50  UnbalancedPower=off  ActivePower=165.711  InductivePower=86.5795  CapacitivePower=0  Pabc=[10e3 9e3 11e3]  QLabc=[100 90 110]  QCabc=[100 90 110]  Pabcp=[10e3 9e3 11e3]  QLabcp=[100 90 110]  QCabcp=[100 90 110]  Measurements=None  LoadType=constant Z
  Load 8733 : spsThreePhaseSeriesRLCLoadLib/Three-Phase Series RLC Load  LConnTagsString=A|B|C  Configuration=Delta  NominalVoltage=11000  Vabc=[1e3 1e3 1e3]  Vabcp=[1e3 1e3 1e3]  NominalFrequency=50  UnbalancedPower=off  ActivePower=5900.5059  InductivePower=2158.2426  CapacitivePower=0  Pabc=[10e3 9e3 11e3]  QLabc=[100 90 110]  QCabc=[100 90 110]  Pabcp=[10e3 9e3 11e3]  QLabcp=[100 90 110]  QCabcp=[100 90 110]  Measurements=None  LoadType=constant Z
  Load 8737 : spsThreePhaseSeriesRLCLoadLib/Three-Phase Series RLC Load  LConnTagsString=A|B|C  Configuration=Delta  NominalVoltage=11000  Vabc=[1e3 1e3 1e3]  Vabcp=[1e3 1e3 1e3]  NominalFrequency=50  UnbalancedPower=off  ActivePower=14045.5122  InductivePower=7263.7158  CapacitivePower=0  Pabc=[10e3 9e3 11e3]  QLabc=[100 90 110]  QCabc=[100 90 110]  Pabcp=[10e3 9e3 11e3]  QLabcp=[100 90 110]  QCabcp=[100 90 110]  Measurements=None  LoadType=constant Z
  Load 9 : spsThreePhaseSeriesRLCLoadLib/Three-Phase Series RLC Load  LConnTagsString=A|B|C  Configuration=Delta  NominalVoltage=11000  Vabc=[1e3 1e3 1e3]  Vabcp=[1e3 1e3 1e3]  NominalFrequency=50  UnbalancedPower=off  ActivePower=5512.4215  InductivePower=2455.2458  CapacitivePower=0  Pabc=[10e3 9e3 11e3]  QLabc=[100 90 110]  QCabc=[100 90 110]  Pabcp=[10e3 9e3 11e3]  QLabcp=[100 90 110]  QCabcp=[100 90 110]  Measurements=None  LoadType=constant Z
  R{1..8} (8 alike) : spsThreePhaseVIMeasurementLib/Three-Phase V-I Measurement  VoltageMeasurement=phase-to-ground  SetLabelV=off  LabelV=Vabc  Vpu=off  VpuLL=off  CurrentMeasurement=yes  SetLabelI=off  LabelI=Iabc  Ipu=off  Pbase=100e6  Vbase=500e3  OutputType=Complex  PhasorSimulation=on  PSBequivalent=0
  Scope R{1..8} (8 alike) : Scope  NumInputPorts=2
  Source PC1_TT2 : spsThreePhaseSourceLib/Three-Phase Source  InternalConnection=Yn  VoltagePhases=off  Voltage=10000  PhaseAngle=0  Voltage_phases=[25e3 25e3 25e3]/sqrt(3)  PhaseAngles_phases=[0 -120 +120]  Frequency=50  NonIdealSource=on  SpecifyImpedance=off  Resistance=0.14  Inductance=0.0031831  ShortCircuitLevel=100e6  BaseVoltage=25e3  XRratio=7  BusType=swing  Pref=10e3  Qref=0  Prefabc=[10e3, 10e3, 10e3]  Qrefabc=[0, 0, 0]  Qmin=-inf  Qmax=inf
  Source Zn : spsSeriesRLCBranchLib/Series RLC Branch  LConnTagsString=__new0  RConnTagsString=__new0  BranchType=RL  Resistance=1e-3  Inductance=3.1831e-06  SetiL0=off  InitialCurrent=0  Capacitance=0  Setx0=off  InitialVoltage=0  Measurements=None
  powergui : spspowerguiLib/powergui  Priority=1  SimulationMode=Phasor  SampleTime=50e-6  frequency=50  Iterations=50  frequencyindice=50  Pbase=100e6  ErrMax=1e-4  UnitsV=kV  UnitsW=MW  buscounter=0  FunctionMessages=off  echomessages=off  EnableUseOfTLC=off  CurrentSourceSwitches=off  DisableSnubberDevices=off  DisableRonSwitches=off  DisableVfSwitches=off  DisplayEquations=off  AutomaticDiscreteSolvers=off  SolverType=Tustin/Backward Euler (TBE)  Interpol=off  ExternalGateDelay=off  methode=off  Ts=10  x0status=blocks  SPID=off  SwTol=0  HookPort=off  NonlinearTolerance=1e-4  nMaxIteration=100  ContinueOnMaxIteration=off  RestoreLinks=warning  ResistiveCurrentMeasurement=off  Frange=[0:2:500]  Ylog=off  Xlog=on  ShowGrid=off  save=off  variable=ZData  structure=0  ZoomFFT=off  StartTime=0.0  cycles=1  DisplayStyle=1  fundamental=60  FreqAxis=off  MaxFrequency=1000  frequencyindicesteady=1  RmsSteady=1  display=off
  wires:
  R5/1 -> Scope R5/1
  R2/2 -> Scope R2/2
  R2/1 -> Scope R2/1
  R5/2 -> Scope R5/2
  R1/2 -> Scope R1/2
  R1/1 -> Scope R1/1
  R3/2 -> Scope R3/2
  R3/1 -> Scope R3/1
  R4/2 -> Scope R4/2
  R4/1 -> Scope R4/1
  R6/1 -> Scope R6/1
  R6/2 -> Scope R6/2
  R7/2 -> Scope R7/2
  R7/1 -> Scope R7/1
  R8/1 -> Scope R8/1
  R8/2 -> Scope R8/2
  connections:
  Source Zn/RConn1 -- Source PC1_TT2/LConn1
  Line 72/LConn1 -- Line 73/RConn1
  Line 72/LConn3 -- Line 73/RConn3
  Line 72/LConn2 -- Line 73/RConn2
  Source Zn/LConn1 -- Ground/LConn1
  Load 28/LConn1 -- Line 108/RConn1
  Line 134/RConn1 -- Line 135/LConn1
  Line 134/RConn3 -- Line 135/LConn3
  Line 134/RConn2 -- Line 135/LConn2
  Load 28/LConn2 -- Line 108/RConn2
  Load 28/LConn3 -- Line 108/RConn3
  Line 182/RConn1 -- Load 56/LConn1
  Line 182/RConn3 -- Load 56/LConn3
  Line 182/RConn2 -- Load 56/LConn2
  Line 69/RConn1 -- Load 8287/LConn1
  Line 69/RConn2 -- Load 8287/LConn2
  Line 69/RConn3 -- Load 8287/LConn3
  Line 55/RConn1 -- Load 8424/LConn1
  Line 55/RConn2 -- Load 8424/LConn2
  Line 55/RConn3 -- Load 8424/LConn3
  Line 42/LConn1 -- Line 40/LConn1 -- Line 43/RConn1
  Line 42/LConn2 -- Line 40/LConn2 -- Line 43/RConn2
  Line 42/LConn3 -- Line 40/LConn3 -- Line 43/RConn3
  Line 159/LConn1 -- Line 158/LConn1 -- Line 157/RConn1
  Line 159/LConn2 -- Line 158/LConn2 -- Line 157/RConn2
  Line 159/LConn3 -- Line 158/LConn3 -- Line 157/RConn3
  Line 146/LConn1 -- Line 145/LConn1 -- Line 96/RConn1
  Line 145/LConn2 -- Line 146/LConn2 -- Line 96/RConn2
  Line 145/LConn3 -- Line 146/LConn3 -- Line 96/RConn3
  Load 16/LConn1 -- Line 204/RConn1
  Load 16/LConn2 -- Line 204/RConn2
  Load 16/LConn3 -- Line 204/RConn3
  Line 89/LConn1 -- Line 88/LConn1 -- Line 149/RConn1
  Line 89/LConn2 -- Line 88/LConn2 -- Line 149/RConn2
  Line 89/LConn3 -- Line 88/LConn3 -- Line 149/RConn3
  Line 148/RConn1 -- Load 49/LConn1
  Line 148/RConn2 -- Load 49/LConn2
  Line 148/RConn3 -- Load 49/LConn3
  Line 58/RConn1 -- Load 8551/LConn1
  Line 58/RConn2 -- Load 8551/LConn2
  Line 58/RConn3 -- Load 8551/LConn3
  Line 152/RConn1 -- Line 163/LConn1
  Line 152/RConn2 -- Line 163/LConn2
  Line 152/RConn3 -- Line 163/LConn3
  Line 119/LConn1 -- Line 120/RConn1 -- Line 118/LConn1
  Line 119/LConn2 -- Line 120/RConn2 -- Line 118/LConn2
  Line 119/LConn3 -- Line 120/RConn3 -- Line 118/LConn3
  Line 158/RConn1 -- Load 42/LConn1
  Line 158/RConn2 -- Load 42/LConn2
  Line 158/RConn3 -- Load 42/LConn3
  Line 198/RConn1 -- Line 199/LConn1
  Line 198/RConn2 -- Line 199/LConn2
  Line 198/RConn3 -- Line 199/LConn3
  Line 84/LConn1 -- Line 41/LConn1 -- Line 85/RConn1
  Line 84/LConn2 -- Line 41/LConn2 -- Line 85/RConn2
  Line 84/LConn3 -- Line 41/LConn3 -- Line 85/RConn3
  Line 192/LConn1 -- Line 191/LConn1 -- Line 195/RConn1
  Line 192/LConn2 -- Line 191/LConn2 -- Line 195/RConn2
  Line 192/LConn3 -- Line 191/LConn3 -- Line 195/RConn3
  Line 121/LConn1 -- Line 120/LConn1 -- Line 126/RConn1
  Line 121/LConn2 -- Line 120/LConn2 -- Line 126/RConn2
  Line 121/LConn3 -- Line 120/LConn3 -- Line 126/RConn3
  Line 54/LConn1 -- Line 53/LConn1 -- Line 59/RConn1
  Line 54/LConn2 -- Line 53/LConn2 -- Line 59/RConn2
  Line 54/LConn3 -- Line 53/LConn3 -- Line 59/RConn3
  Load 39/LConn1 -- Line 119/RConn1
  Load 39/LConn2 -- Line 119/RConn2
  Load 39/LConn3 -- Line 119/RConn3
  Line 23/LConn1 -- Line 22/LConn1 -- Line 24/RConn1
  Line 23/LConn2 -- Line 22/LConn2 -- Line 24/RConn2
  Line 23/LConn3 -- Line 22/LConn3 -- Line 24/RConn3
  Line 2/RConn1 -- R4/LConn1
  Line 2/RConn2 -- R4/LConn2
  Line 2/RConn3 -- R4/LConn3
  Line 132/LConn1 -- Line 131/LConn1 -- Line 133/RConn1
  Line 132/LConn2 -- Line 131/LConn2 -- Line 133/RConn2
  Line 132/LConn3 -- Line 131/LConn3 -- Line 133/RConn3
  Line 12/RConn1 -- Load 31/LConn1
  Line 12/RConn2 -- Load 31/LConn2
  Line 12/RConn3 -- Load 31/LConn3
  Load 32/LConn1 -- Line 5/LConn1 -- Line 6/RConn1
  Load 32/LConn2 -- Line 5/LConn2 -- Line 6/RConn2
  Load 32/LConn3 -- Line 5/LConn3 -- Line 6/RConn3
  Line 161/LConn1 -- Line 160/LConn1 -- Line im7/RConn1
  Line 161/LConn2 -- Line 160/LConn2 -- Line im7/RConn2
  Line 161/LConn3 -- Line 160/LConn3 -- Line im7/RConn3
  Line 101/LConn1 -- Line 100/LConn1 -- Line 99/RConn1
  Line 101/LConn2 -- Line 100/LConn2 -- Line 99/RConn2
  Line 101/LConn3 -- Line 100/LConn3 -- Line 99/RConn3
  Line 103/RConn1 -- Line 104/LConn1
  Line 103/RConn2 -- Line 104/LConn2
  Line 103/RConn3 -- Line 104/LConn3
  Line 74/LConn1 -- R2/RConn1
  Line 74/LConn2 -- R2/RConn2
  Line 74/LConn3 -- R2/RConn3
  Line 164/RConn1 -- R8/LConn1
  Line 164/RConn2 -- R8/LConn2
  Line 164/RConn3 -- R8/LConn3
  Line 168/LConn1 -- Line 169/RConn1
  Line 168/LConn2 -- Line 169/RConn2
  Line 168/LConn3 -- Line 169/RConn3
  Line 68/LConn1 -- Line 67/LConn1 -- Line 70/RConn1
  Line 68/LConn2 -- Line 67/LConn2 -- Line 70/RConn2
  Line 68/LConn3 -- Line 67/LConn3 -- Line 70/RConn3
  Line 44/LConn1 -- Line 45/RConn1
  Line 44/LConn2 -- Line 45/RConn2
  Line 44/LConn3 -- Line 45/RConn3
  Line 203/RConn1 -- Line 202/LConn1
  Line 203/RConn2 -- Line 202/LConn2
  Line 203/RConn3 -- Line 202/LConn3
  Line 14/RConn1 -- Load 30/LConn1
  Line 14/RConn2 -- Load 30/LConn2
  Line 14/RConn3 -- Load 30/LConn3
  Line 10/LConn1 -- Line 11/LConn1 -- Line 16/RConn1
  Line 11/LConn2 -- Line 10/LConn2 -- Line 16/RConn2
  Line 11/LConn3 -- Line 10/LConn3 -- Line 16/RConn3
  Line 103/LConn1 -- Line 102/LConn1 -- Line im5/RConn1
  Line 103/LConn2 -- Line 102/LConn2 -- Line im5/RConn2
  Line 103/LConn3 -- Line 102/LConn3 -- Line im5/RConn3
  Line 71/LConn1 -- Line 70/LConn1 -- Line 72/RConn1
  Line 71/LConn2 -- Line 70/LConn2 -- Line 72/RConn2
  Line 71/LConn3 -- Line 70/LConn3 -- Line 72/RConn3
  Line 4/LConn1 -- Line 2/LConn1 -- Line 5/RConn1
  Line 4/LConn2 -- Line 2/LConn2 -- Line 5/RConn2
  Line 4/LConn3 -- Line 2/LConn3 -- Line 5/RConn3
  Line 7/LConn1 -- Line 6/LConn1 -- Line 8/RConn1
  Line 7/LConn2 -- Line 6/LConn2 -- Line 8/RConn2
  Line 7/LConn3 -- Line 6/LConn3 -- Line 8/RConn3
  Line 60/RConn1 -- Line 61/LConn1
  Line 60/RConn2 -- Line 61/LConn2
  Line 60/RConn3 -- Line 61/LConn3
  Line 15/RConn1 -- Load 33/LConn1
  Line 15/RConn2 -- Load 33/LConn2
  Line 15/RConn3 -- Load 33/LConn3
  Load 13/LConn1 -- Line 205/RConn1
  Load 13/LConn2 -- Line 205/RConn2
  Load 13/LConn3 -- Line 205/RConn3
  Line 200/LConn1 -- Line 201/LConn1 -- Line 199/RConn1
  Line 201/LConn2 -- Line 200/LConn2 -- Line 199/RConn2
  Line 200/LConn3 -- Line 201/LConn3 -- Line 199/RConn3
  Line 23/RConn1 -- Load 8/LConn1
  Line 23/RConn2 -- Load 8/LConn2
  Line 23/RConn3 -- Load 8/LConn3
  Load 5/LConn1 -- Line 146/RConn1
  Load 5/LConn2 -- Line 146/RConn2
  Load 5/LConn3 -- Line 146/RConn3
  Line 36/LConn1 -- Line 35/LConn1 -- Line 34/RConn1
  Line 36/LConn2 -- Line 35/LConn2 -- Line 34/RConn2
  Line 36/LConn3 -- Line 35/LConn3 -- Line 34/RConn3
  Load 9/LConn1 -- Line 20/RConn1
  Load 9/LConn2 -- Line 20/RConn2
  Load 9/LConn3 -- Line 20/RConn3
  Line 129/RConn1 -- Line 93/LConn3
  Line 129/RConn2 -- Line 93/LConn2
  Line 129/RConn3 -- Line 93/LConn1
  Line 56/LConn1 -- Line 55/LConn1 -- Line 54/RConn1
  Line 56/LConn2 -- Line 55/LConn2 -- Line 54/RConn2
  Line 56/LConn3 -- Line 55/LConn3 -- Line 54/RConn3
  Line 135/RConn1 -- Load 21/LConn1
  Line 135/RConn2 -- Load 21/LConn2
  Line 135/RConn3 -- Load 21/LConn3
  Line 51/LConn1 -- Line 52/LConn1 -- Line 53/RConn1
  Line 51/LConn2 -- Line 52/LConn2 -- Line 53/RConn2
  Line 51/LConn3 -- Line 52/LConn3 -- Line 53/RConn3
  Line 134/LConn1 -- Line 133/LConn1 -- Line 137/RConn1
  Line 134/LConn2 -- Line 133/LConn2 -- Line 137/RConn2
  Line 134/LConn3 -- Line 133/LConn3 -- Line 137/RConn3
  Line 115/LConn1 -- Line 114/LConn1 -- Line 113/RConn1
  Line 115/LConn2 -- Line 114/LConn2 -- Line 113/RConn2
  Line 115/LConn3 -- Line 114/LConn3 -- Line 113/RConn3
  Load 6/LConn1 -- Line 21/LConn1 -- Line 22/RConn1
  Load 6/LConn2 -- Line 21/LConn2 -- Line 22/RConn2
  Load 6/LConn3 -- Line 21/LConn3 -- Line 22/RConn3
  Load 52/LConn1 -- Line 85/LConn1 -- Line 86/RConn1
  Load 52/LConn2 -- Line 85/LConn2 -- Line 86/RConn2
  Load 52/LConn3 -- Line 85/LConn3 -- Line 86/RConn3
  Line 152/LConn1 -- Load 47/LConn1 -- Line 188/RConn1 -- Line 83/LConn1
  Line 152/LConn2 -- Load 47/LConn2 -- Line 83/LConn2 -- Line 188/RConn2
  Line 152/LConn3 -- Load 47/LConn3 -- Line 188/RConn3 -- Line 83/LConn3
  Line 49/LConn1 -- Line 48/LConn1 -- Line 47/RConn1
  Line 49/LConn2 -- Line 48/LConn2 -- Line 47/RConn2
  Line 49/LConn3 -- Line 48/LConn3 -- Line 47/RConn3
  Line 125/LConn1 -- Line 124/LConn1 -- Line 123/RConn1
  Line 125/LConn2 -- Line 124/LConn2 -- Line 123/RConn2
  Line 125/LConn3 -- Line 124/LConn3 -- Line 123/RConn3
  Line 124/RConn1 -- Load 36/LConn1
  Line 124/RConn2 -- Load 36/LConn2
  Line 124/RConn3 -- Load 36/LConn3
  Source PC1_TT2/RConn1 -- R2/LConn1
  Source PC1_TT2/RConn2 -- R2/LConn2
  Source PC1_TT2/RConn3 -- R2/LConn3
  Line 196/LConn1 -- Line 195/LConn1 -- Line 197/RConn1
  Line 196/LConn2 -- Line 195/LConn2 -- Line 197/RConn2
  Line 196/LConn3 -- Line 195/LConn3 -- Line 197/RConn3
  Line 166/LConn1 -- Line 164/LConn1 -- Line 167/RConn1
  Line 166/LConn2 -- Line 164/LConn2 -- Line 167/RConn2
  Line 166/LConn3 -- Line 164/LConn3 -- Line 167/RConn3
  Line 25/RConn1 -- Line 26/LConn1
  Line 25/RConn2 -- Line 26/LConn2
  Line 25/RConn3 -- Line 26/LConn3
  Load 35/LConn1 -- Line 117/RConn1 -- Line 111/LConn1 -- Line 112/LConn1
  Load 35/LConn2 -- Line 117/RConn2 -- Line 111/LConn2 -- Line 112/LConn2
  Load 35/LConn3 -- Line 117/RConn3 -- Line 111/LConn3 -- Line 112/LConn3
  Line 196/RConn1 -- Load 15/LConn1
  Line 196/RConn2 -- Load 15/LConn2
  Line 196/RConn3 -- Load 15/LConn3
  Line 112/RConn1 -- Line 113/LConn1
  Line 112/RConn2 -- Line 113/LConn2
  Line 112/RConn3 -- Line 113/LConn3
  Line 187/RConn1 -- Line 151/LConn3
  Line 187/RConn2 -- Line 151/LConn2
  Line 187/RConn3 -- Line 151/LConn1
  Load 60/LConn1 -- Line 84/RConn1
  Load 60/LConn2 -- Line 84/RConn2
  Load 60/LConn3 -- Line 84/RConn3
  Load 48/LConn1 -- Line 166/RConn1
  Load 48/LConn2 -- Line 166/RConn2
  Load 48/LConn3 -- Line 166/RConn3
  Line 57/RConn1 -- Load 8293/LConn1
  Line 57/RConn2 -- Load 8293/LConn2
  Line 57/RConn3 -- Load 8293/LConn3
  Line 136/RConn1 -- Line 130/LConn1
  Line 136/RConn2 -- Line 130/LConn2
  Line 136/RConn3 -- Line 130/LConn3
  Line 147/LConn1 -- Line 136/LConn1 -- Line 10/RConn1
  Line 147/LConn2 -- Line 136/LConn2 -- Line 10/RConn2
  Line 136/LConn3 -- Line 147/LConn3 -- Line 10/RConn3
  Line 87/LConn1 -- Line 86/LConn1 -- Line 88/RConn1
  Line 87/LConn2 -- Line 86/LConn2 -- Line 88/RConn2
  Line 87/LConn3 -- Line 86/LConn3 -- Line 88/RConn3
  Load 7/LConn1 -- Line 144/RConn1 -- Line 140/LConn1 -- Line 107/LConn1
  Line 140/LConn2 -- Load 7/LConn2 -- Line 107/LConn2 -- Line 144/RConn2
  Load 7/LConn3 -- Line 107/LConn3 -- Line 140/LConn3 -- Line 144/RConn3
  Line 79/RConn1 -- Load 14/LConn1
  Line 79/RConn2 -- Load 14/LConn2
  Line 79/RConn3 -- Load 14/LConn3
  Line 1/LConn1 -- Line 3/RConn1
  Line 1/LConn2 -- Line 3/RConn2
  Line 1/LConn3 -- Line 3/RConn3
  Line 33/RConn1 -- Load 51/LConn1
  Line 33/RConn2 -- Load 51/LConn2
  Line 33/RConn3 -- Load 51/LConn3
  Line 186/RConn1 -- Line 187/LConn1
  Line 186/RConn2 -- Line 187/LConn2
  Line 186/RConn3 -- Line 187/LConn3
  Line 89/RConn1 -- Line 148/LConn1
  Line 89/RConn2 -- Line 148/LConn2
  Line 89/RConn3 -- Line 148/LConn3
  Line im3/LConn1 -- R5/RConn1
  Line im3/LConn2 -- R5/RConn2
  Line im3/LConn3 -- R5/RConn3
  Line 181/LConn1 -- Line 180/LConn1 -- Line 179/RConn1
  Line 181/LConn2 -- Line 180/LConn2 -- Line 179/RConn2
  Line 181/LConn3 -- Line 180/LConn3 -- Line 179/RConn3
  Line 95/LConn1 -- Line 107/RConn1
  Line 95/LConn2 -- Line 107/RConn2
  Line 95/LConn3 -- Line 107/RConn3
  Line 81/RConn1 -- Load 11/LConn1
  Line 81/RConn2 -- Load 11/LConn2
  Line 81/RConn3 -- Load 11/LConn3
  Line 177/LConn1 -- Line 178/RConn1 -- Line 176/LConn1
  Line 177/LConn2 -- Line 178/RConn2 -- Line 176/LConn2
  Line 177/LConn3 -- Line 178/RConn3 -- Line 176/LConn3
  Load 20/LConn1 -- Line 42/RConn1
  Load 20/LConn2 -- Line 42/RConn2
  Load 20/LConn3 -- Line 42/RConn3
  Line 183/LConn1 -- Line 182/LConn1 -- Line 181/RConn1
  Line 183/LConn2 -- Line 182/LConn2 -- Line 181/RConn2
  Line 183/LConn3 -- Line 182/LConn3 -- Line 181/RConn3
  Line 49/RConn1 -- Line 82/LConn1
  Line 49/RConn2 -- Line 82/LConn2
  Line 49/RConn3 -- Line 82/LConn3
  Line 183/RConn1 -- Load 58/LConn1
  Line 183/RConn2 -- Load 58/LConn2
  Line 183/RConn3 -- Load 58/LConn3
  Line 30/LConn1 -- Line 83/RConn1
  Line 30/LConn2 -- Line 83/RConn2
  Line 30/LConn3 -- Line 83/RConn3
  Line 132/RConn1 -- Load 26/LConn1
  Line 132/RConn2 -- Load 26/LConn2
  Line 132/RConn3 -- Load 26/LConn3
  Line 61/RConn1 -- Line 29/LConn3
  Line 61/RConn2 -- Line 29/LConn2
  Line 61/RConn3 -- Line 29/LConn1
  Line 122/RConn1 -- Load 37/LConn1
  Line 122/RConn2 -- Load 37/LConn2
  Line 122/RConn3 -- Load 37/LConn3
  Line 204/LConn1 -- Line 203/LConn1 -- Line 154/RConn1
  Line 203/LConn2 -- Line 204/LConn2 -- Line 154/RConn2
  Line 203/LConn3 -- Line 204/LConn3 -- Line 154/RConn3
  Line 106/RConn1 -- R6/LConn1
  Line 106/RConn2 -- R6/LConn2
  Line 106/RConn3 -- R6/LConn3
  Line im2/LConn1 -- R3/RConn1
  Line im2/LConn2 -- R3/RConn2
  Line im2/LConn3 -- R3/RConn3
  Line 150/RConn1 -- Load 12/LConn1
  Line 150/RConn2 -- Load 12/LConn2
  Line 150/RConn3 -- Load 12/LConn3
  Line im1/LConn1 -- R1/RConn1
  Line im1/LConn2 -- R1/RConn2
  Line im1/LConn3 -- R1/RConn3
  Line 15/LConn1 -- Line 14/LConn1 -- Line 13/RConn1
  Line 15/LConn2 -- Line 14/LConn2 -- Line 13/RConn2
  Line 15/LConn3 -- Line 14/LConn3 -- Line 13/RConn3
  Line 190/LConn1 -- Line 189/LConn1 -- Line 191/RConn1
  Line 190/LConn2 -- Line 189/LConn2 -- Line 191/RConn2
  Line 190/LConn3 -- Line 189/LConn3 -- Line 191/RConn3
  Line 176/RConn1 -- Line 175/LConn1
  Line 176/RConn2 -- Line 175/LConn2
  Line 176/RConn3 -- Line 175/LConn3
  Line 66/LConn1 -- Line 65/LConn1 -- Line 67/RConn1
  Line 66/LConn2 -- Line 65/LConn2 -- Line 67/RConn2
  Line 66/LConn3 -- Line 65/LConn3 -- Line 67/RConn3
  Line 140/RConn1 -- Line 141/LConn1
  Line 140/RConn2 -- Line 141/LConn2
  Line 140/RConn3 -- Line 141/LConn3
  Line 159/RConn1 -- Load 45/LConn1
  Line 159/RConn2 -- Load 45/LConn2
  Line 159/RConn3 -- Load 45/LConn3
  Line 100/RConn1 -- Load 22/LConn1
  Line 100/RConn2 -- Load 22/LConn2
  Line 100/RConn3 -- Load 22/LConn3
  Line 87/RConn1 -- Load 54/LConn1
  Line 87/RConn2 -- Load 54/LConn2
  Line 87/RConn3 -- Load 54/LConn3
  Line 127/LConn1 -- Line 116/LConn1 -- Line 105/RConn1
  Line 127/LConn2 -- Line 116/LConn2 -- Line 105/RConn2
  Line 116/LConn3 -- Line 127/LConn3 -- Line 105/RConn3
  Load 8733/LConn1 -- Line 63/RConn1
  Load 8733/LConn2 -- Line 63/RConn2
  Load 8733/LConn3 -- Line 63/RConn3
  Line 155/LConn1 -- Line 154/LConn1 -- Line 160/RConn1
  Line 155/LConn2 -- Line 154/LConn2 -- Line 160/RConn2
  Line 155/LConn3 -- Line 154/LConn3 -- Line 160/RConn3
  Line 73/LConn1 -- Line 74/RConn1
  Line 73/LConn2 -- Line 74/RConn2
  Line 73/LConn3 -- Line 74/RConn3
  Line 126/LConn3 -- Line 128/LConn3 -- Line im1/RConn1
  Line 126/LConn2 -- Line 128/LConn2 -- Line im1/RConn2
  Line 126/LConn1 -- Line 128/LConn1 -- Line im1/RConn3
  Line 76/RConn1 -- Load 19/LConn1
  Line 76/RConn2 -- Load 19/LConn2
  Line 76/RConn3 -- Load 19/LConn3
  Line 170/LConn1 -- Load 55/LConn1 -- Line 175/RConn1 -- Line 169/LConn1
  Line 170/LConn2 -- Load 55/LConn2 -- Line 175/RConn2 -- Line 169/LConn2
  Line 170/LConn3 -- Load 55/LConn3 -- Line 175/RConn3 -- Line 169/LConn3
  Line 173/LConn1 -- Line 172/LConn1 -- Line 171/RConn1
  Line 173/LConn2 -- Line 172/LConn2 -- Line 171/RConn2
  Line 173/LConn3 -- Line 172/LConn3 -- Line 171/RConn3
  Line 128/RConn1 -- Line 129/LConn1
  Line 128/RConn2 -- Line 129/LConn2
  Line 128/RConn3 -- Line 129/LConn3
  Line 25/LConn1 -- Line 24/LConn1 -- Line 27/RConn1
  Line 25/LConn2 -- Line 24/LConn2 -- Line 27/RConn2
  Line 25/LConn3 -- Line 24/LConn3 -- Line 27/RConn3
  Load 40/LConn1 -- Line 4/RConn1
  Load 40/LConn2 -- Line 4/RConn2
  Load 40/LConn3 -- Line 4/RConn3
  Line 9/LConn1 -- Line 8/LConn1 -- Line 91/RConn1
  Line 9/LConn2 -- Line 8/LConn2 -- Line 91/RConn2
  Line 9/LConn3 -- Line 8/LConn3 -- Line 91/RConn3
  Line 13/LConn1 -- Line 12/LConn1 -- Line 11/RConn1
  Line 13/LConn2 -- Line 12/LConn2 -- Line 11/RConn2
  Line 13/LConn3 -- Line 12/LConn3 -- Line 11/RConn3
  Line 94/RConn1 -- Line 105/LConn1
  Line 94/RConn2 -- Line 105/LConn2
  Line 94/RConn3 -- Line 105/LConn3
  Line 78/LConn1 -- Line 77/LConn1 -- Line 80/RConn1
  Line 78/LConn2 -- Line 77/LConn2 -- Line 80/RConn2
  Line 78/LConn3 -- Line 77/LConn3 -- Line 80/RConn3
  Load 27/LConn1 -- Line 94/LConn1 -- Line 3/LConn1 -- Line 130/RConn1
  Line 3/LConn2 -- Line 94/LConn2 -- Line 130/RConn2 -- Load 27/LConn2
  Load 27/LConn3 -- Line 94/LConn3 -- Line 3/LConn3 -- Line 130/RConn3
  Line 157/LConn1 -- Line 156/LConn1 -- Line 155/RConn1
  Line 157/LConn2 -- Line 156/LConn2 -- Line 155/RConn2
  Line 157/LConn3 -- Line 156/LConn3 -- Line 155/RConn3
  Line 118/RConn1 -- Line 117/LConn1
  Line 118/RConn2 -- Line 117/LConn2
  Line 118/RConn3 -- Line 117/LConn3
  Load 8485/LConn1 -- Line 64/LConn1 -- Line 65/RConn1
  Load 8485/LConn2 -- Line 64/LConn2 -- Line 65/RConn2
  Load 8485/LConn3 -- Line 64/LConn3 -- Line 65/RConn3
  Line 185/LConn1 -- Line 174/LConn1 -- Line 163/RConn1
  Line 185/LConn2 -- Line 174/LConn2 -- Line 163/RConn2
  Line 174/LConn3 -- Line 185/LConn3 -- Line 163/RConn3
  Load 8737/LConn1 -- Line 52/RConn1
  Load 8737/LConn2 -- Line 52/RConn2
  Load 8737/LConn3 -- Line 52/RConn3
  Line 36/RConn1 -- Load 53/LConn1
  Line 36/RConn2 -- Load 53/LConn2
  Line 36/RConn3 -- Load 53/LConn3
  Line 66/RConn1 -- Load 8605/LConn1
  Line 66/RConn2 -- Load 8605/LConn2
  Line 66/RConn3 -- Load 8605/LConn3
  Line 153/LConn1 -- Line 165/RConn1
  Line 153/LConn2 -- Line 165/RConn2
  Line 153/LConn3 -- Line 165/RConn3
  Line 123/LConn1 -- Line 122/LConn1 -- Line 121/RConn1
  Line 123/LConn2 -- Line 122/LConn2 -- Line 121/RConn2
  Line 123/LConn3 -- Line 122/LConn3 -- Line 121/RConn3
  Line 9/RConn1 -- Line 90/LConn1
  Line 9/RConn2 -- Line 90/LConn2
  Line 9/RConn3 -- Line 90/LConn3
  Line 165/LConn1 -- Line 198/LConn1 -- Line 202/RConn1 -- Load 18/LConn1
  Line 198/LConn2 -- Line 165/LConn2 -- Load 18/LConn2 -- Line 202/RConn2
  Load 18/LConn3 -- Line 198/LConn3 -- Line 165/LConn3 -- Line 202/RConn3
  Line 108/LConn1 -- Line 106/LConn1 -- Line 109/RConn1
  Line 108/LConn2 -- Line 106/LConn2 -- Line 109/RConn2
  Line 108/LConn3 -- Line 106/LConn3 -- Line 109/RConn3
  Line 138/LConn1 -- Line 137/LConn1 -- Line 139/RConn1
  Line 138/LConn2 -- Line 137/LConn2 -- Line 139/RConn2
  Line 138/LConn3 -- Line 137/LConn3 -- Line 139/RConn3
  Load 10/LConn1 -- Line 147/RConn1
  Load 10/LConn2 -- Line 147/RConn2
  Load 10/LConn3 -- Line 147/RConn3
  Line 7/RConn1 -- Load 34/LConn1
  Line 7/RConn2 -- Load 34/LConn2
  Line 7/RConn3 -- Load 34/LConn3
  Line 31/LConn1 -- Line 32/LConn1 -- Line 37/RConn1
  Line 32/LConn2 -- Line 31/LConn2 -- Line 37/RConn2
  Line 32/LConn3 -- Line 31/LConn3 -- Line 37/RConn3
  Line 110/LConn1 -- Line 111/RConn1
  Line 110/LConn2 -- Line 111/RConn2
  Line 110/LConn3 -- Line 111/RConn3
  Line im4/LConn1 -- R4/RConn1
  Line im4/LConn2 -- R4/RConn2
  Line im4/LConn3 -- R4/RConn3
  Line 20/LConn1 -- Line 19/LConn1 -- Line 21/RConn1
  Line 20/LConn2 -- Line 19/LConn2 -- Line 21/RConn2
  Line 20/LConn3 -- Line 19/LConn3 -- Line 21/RConn3
  Line 28/RConn1 -- Load 1/LConn1
  Line 28/RConn2 -- Load 1/LConn2
  Line 28/RConn3 -- Load 1/LConn3
  Line 92/RConn1 -- Load 2/LConn1
  Line 92/RConn2 -- Load 2/LConn2
  Line 92/RConn3 -- Load 2/LConn3
  Line 101/RConn1 -- Load 25/LConn1
  Line 101/RConn2 -- Load 25/LConn2
  Line 101/RConn3 -- Load 25/LConn3
  Line 28/LConn1 -- Line 27/LConn1 -- Line 29/RConn1
  Line 28/LConn2 -- Line 27/LConn2 -- Line 29/RConn2
  Line 28/LConn3 -- Line 27/LConn3 -- Line 29/RConn3
  Load 24/LConn1 -- Line 109/LConn1 -- Line 131/RConn1
  Load 24/LConn2 -- Line 109/LConn2 -- Line 131/RConn2
  Load 24/LConn3 -- Line 109/LConn3 -- Line 131/RConn3
  Line 194/RConn1 -- Line 188/LConn1
  Line 194/RConn2 -- Line 188/LConn2
  Line 194/RConn3 -- Line 188/LConn3
  Line 90/RConn1 -- Load 29/LConn1
  Line 90/RConn2 -- Load 29/LConn2
  Line 90/RConn3 -- Load 29/LConn3
  Line 173/RConn1 -- Line 197/LConn1
  Line 173/RConn2 -- Line 197/LConn2
  Line 173/RConn3 -- Line 197/LConn3
  Load 44/LConn1 -- Line 167/LConn1 -- Line 189/RConn1
  Load 44/LConn2 -- Line 167/LConn2 -- Line 189/RConn2
  Load 44/LConn3 -- Line 167/LConn3 -- Line 189/RConn3
  Line 41/RConn1 -- R7/LConn1
  Line 41/RConn2 -- R7/LConn2
  Line 41/RConn3 -- R7/LConn3
  Line 35/RConn1 -- Load 50/LConn1
  Line 35/RConn2 -- Load 50/LConn2
  Line 35/RConn3 -- Load 50/LConn3
  Line 40/RConn1 -- R3/LConn1
  Line 40/RConn2 -- R3/LConn2
  Line 40/RConn3 -- R3/LConn3
  Load 59/LConn1 -- Line 177/RConn1
  Load 59/LConn2 -- Line 177/RConn2
  Load 59/LConn3 -- Line 177/RConn3
  Line 145/RConn1 -- Line 144/LConn1
  Line 145/RConn2 -- Line 144/LConn2
  Line 145/RConn3 -- Line 144/LConn3
  Line 58/LConn1 -- Line 57/LConn1 -- Line 56/RConn1
  Line 58/LConn2 -- Line 57/LConn2 -- Line 56/RConn2
  Line 58/LConn3 -- Line 57/LConn3 -- Line 56/RConn3
  Line im6/LConn1 -- R7/RConn1
  Line im6/LConn2 -- R7/RConn2
  Line im6/LConn3 -- R7/RConn3
  Line 193/RConn1 -- Load 41/LConn1
  Line 193/RConn2 -- Load 41/LConn2
  Line 193/RConn3 -- Load 41/LConn3
  Line 180/RConn1 -- Load 57/LConn1
  Line 180/RConn2 -- Load 57/LConn2
  Line 180/RConn3 -- Load 57/LConn3
  Line 81/LConn1 -- Line 80/LConn1 -- Line 82/RConn1
  Line 81/LConn2 -- Line 80/LConn2 -- Line 82/RConn2
  Line 81/LConn3 -- Line 80/LConn3 -- Line 82/RConn3
  Line 59/LConn1 -- Line im3/RConn1 -- Line 60/LConn1
  Line 59/LConn2 -- Line im3/RConn2 -- Line 60/LConn2
  Line 59/LConn3 -- Line im3/RConn3 -- Line 60/LConn3
  Line 205/LConn1 -- Line 194/LConn1 -- Line 31/RConn1
  Line 194/LConn2 -- Line 205/LConn2 -- Line 31/RConn2
  Line 205/LConn3 -- Line 194/LConn3 -- Line 31/RConn3
  Line 34/LConn1 -- Line 33/LConn1 -- Line 32/RConn1
  Line 34/LConn2 -- Line 33/LConn2 -- Line 32/RConn2
  Line 34/LConn3 -- Line 33/LConn3 -- Line 32/RConn3
  Line im5/LConn1 -- R6/RConn1
  Line im5/LConn2 -- R6/RConn2
  Line im5/LConn3 -- R6/RConn3
  Line 17/RConn1 -- Line 18/LConn1
  Line 17/RConn2 -- Line 18/LConn2
  Line 17/RConn3 -- Line 18/LConn3
  Line 71/RConn1 -- Load 8041/LConn1
  Line 71/RConn2 -- Load 8041/LConn2
  Line 71/RConn3 -- Load 8041/LConn3
  Line 45/LConn1 -- Line 46/LConn1 -- Load 8173/LConn1 -- Line 50/RConn1
  Line 45/LConn2 -- Line 46/LConn2 -- Load 8173/LConn2 -- Line 50/RConn2
  Line 45/LConn3 -- Line 46/LConn3 -- Load 8173/LConn3 -- Line 50/RConn3
  Line 68/RConn1 -- Line 69/LConn1
  Line 68/RConn2 -- Line 69/LConn2
  Line 68/RConn3 -- Line 69/LConn3
  Line 19/RConn1 -- R1/LConn1
  Line 19/RConn2 -- R1/LConn2
  Line 19/RConn3 -- R1/LConn3
  Line 125/RConn1 -- Load 38/LConn1
  Line 125/RConn2 -- Load 38/LConn2
  Line 125/RConn3 -- Load 38/LConn3
  Line im7/LConn1 -- R8/RConn1
  Line im7/LConn2 -- R8/RConn2
  Line im7/LConn3 -- R8/RConn3
  Line 38/RConn1 -- Line 39/LConn1
  Line 38/RConn2 -- Line 39/LConn2
  Line 38/RConn3 -- Line 39/LConn3
  Line 62/RConn1 -- R5/LConn1
  Line 62/RConn2 -- R5/LConn2
  Line 62/RConn3 -- R5/LConn3
  Line 78/RConn1 -- Line 79/LConn1
  Line 78/RConn2 -- Line 79/LConn2
  Line 78/RConn3 -- Line 79/LConn3
  Line 76/LConn1 -- Line 75/LConn1 -- Line 77/RConn1
  Line 76/LConn2 -- Line 75/LConn2 -- Line 77/RConn2
  Line 76/LConn3 -- Line 75/LConn3 -- Line 77/RConn3
  Load 17/LConn1 -- Line 43/LConn1 -- Line 75/RConn1
  Load 17/LConn2 -- Line 43/LConn2 -- Line 75/RConn2
  Load 17/LConn3 -- Line 43/LConn3 -- Line 75/RConn3
  Line 190/RConn1 -- Load 46/LConn1
  Line 190/RConn2 -- Load 46/LConn2
  Line 190/RConn3 -- Load 46/LConn3
  Line 97/LConn1 -- Line 96/LConn1 -- Line 102/RConn1
  Line 97/LConn2 -- Line 96/LConn2 -- Line 102/RConn2
  Line 97/LConn3 -- Line 96/LConn3 -- Line 102/RConn3
  Line 170/RConn1 -- Line 171/LConn1
  Line 170/RConn2 -- Line 171/LConn2
  Line 170/RConn3 -- Line 171/LConn3
  Line 186/LConn1 -- Line 184/LConn1 -- Line im2/RConn1
  Line 186/LConn2 -- Line 184/LConn2 -- Line im2/RConn2
  Line 186/LConn3 -- Line 184/LConn3 -- Line im2/RConn3
  Line 38/LConn1 -- Line 37/LConn1 -- Line im6/RConn1
  Line 38/LConn2 -- Line 37/LConn2 -- Line im6/RConn2
  Line 38/LConn3 -- Line im6/RConn3 -- Line 37/LConn3
  Line 16/LConn1 -- Line 17/LConn1 -- Line im4/RConn1
  Line 16/LConn2 -- Line 17/LConn2 -- Line im4/RConn2
  Line 16/LConn3 -- Line 17/LConn3 -- Line im4/RConn3
  Line 98/RConn1 -- Load 23/LConn1
  Line 98/RConn2 -- Load 23/LConn2
  Line 98/RConn3 -- Load 23/LConn3
  Line 179/LConn1 -- Line 178/LConn1 -- Line 184/RConn1
  Line 179/LConn2 -- Line 178/LConn2 -- Line 184/RConn2
  Line 179/LConn3 -- Line 178/LConn3 -- Line 184/RConn3
  Line 51/RConn1 -- Line 50/LConn1
  Line 51/RConn2 -- Line 50/LConn2
  Line 51/RConn3 -- Line 50/LConn3
  Line 192/RConn1 -- Line 193/LConn1
  Line 192/RConn2 -- Line 193/LConn2
  Line 192/RConn3 -- Line 193/LConn3
  Line 156/RConn1 -- Load 43/LConn1
  Line 156/RConn2 -- Load 43/LConn2
  Line 156/RConn3 -- Load 43/LConn3
  Line 142/LConn1 -- Line 143/LConn1 -- Line 141/RConn1
  Line 143/LConn2 -- Line 142/LConn2 -- Line 141/RConn2
  Line 142/LConn3 -- Line 143/LConn3 -- Line 141/RConn3
  Line 115/RConn1 -- Line 139/LConn1
  Line 115/RConn2 -- Line 139/LConn2
  Line 115/RConn3 -- Line 139/LConn3
  Line 46/RConn1 -- Line 47/LConn1
  Line 46/RConn2 -- Line 47/LConn2
  Line 46/RConn3 -- Line 47/LConn3
  Line 26/RConn1 -- Load 3/LConn1
  Line 26/RConn2 -- Load 3/LConn2
  Line 26/RConn3 -- Load 3/LConn3
  Line 138/RConn1 -- Load 4/LConn1
  Line 138/RConn2 -- Load 4/LConn2
  Line 138/RConn3 -- Load 4/LConn3
  Line 63/LConn1 -- Line 62/LConn1 -- Line 64/RConn1
  Line 63/LConn2 -- Line 62/LConn2 -- Line 64/RConn2
  Line 63/LConn3 -- Line 62/LConn3 -- Line 64/RConn3
  Line 150/LConn1 -- Line 149/LConn1 -- Line 151/RConn1
  Line 150/LConn2 -- Line 149/LConn2 -- Line 151/RConn2
  Line 150/LConn3 -- Line 149/LConn3 -- Line 151/RConn3
  Line 92/LConn1 -- Line 91/LConn1 -- Line 93/RConn1
  Line 92/LConn2 -- Line 91/LConn2 -- Line 93/RConn2
  Line 92/LConn3 -- Line 91/LConn3 -- Line 93/RConn3
  Line 161/RConn1 -- Line 162/LConn1
  Line 161/RConn2 -- Line 162/LConn2
  Line 161/RConn3 -- Line 162/LConn3
  Line 99/LConn1 -- Line 98/LConn1 -- Line 97/RConn1
  Line 99/LConn2 -- Line 98/LConn2 -- Line 97/RConn2
  Line 99/LConn3 -- Line 98/LConn3 -- Line 97/RConn3
